simulink model "c00003M_harness"  (R2018a)
settings: Solver=FixedStepAuto  StartTime=0.0  StopTime=300  FixedStep=0.1  RelTol=1e-3
undefined symbols (not defined in the file): A1, hmax, PriorityTank, R1, R2, sigbuilder_block
(part 1 of 44)
settings Model: Creator=aarrieta  LastModifiedBy=umarkiegi

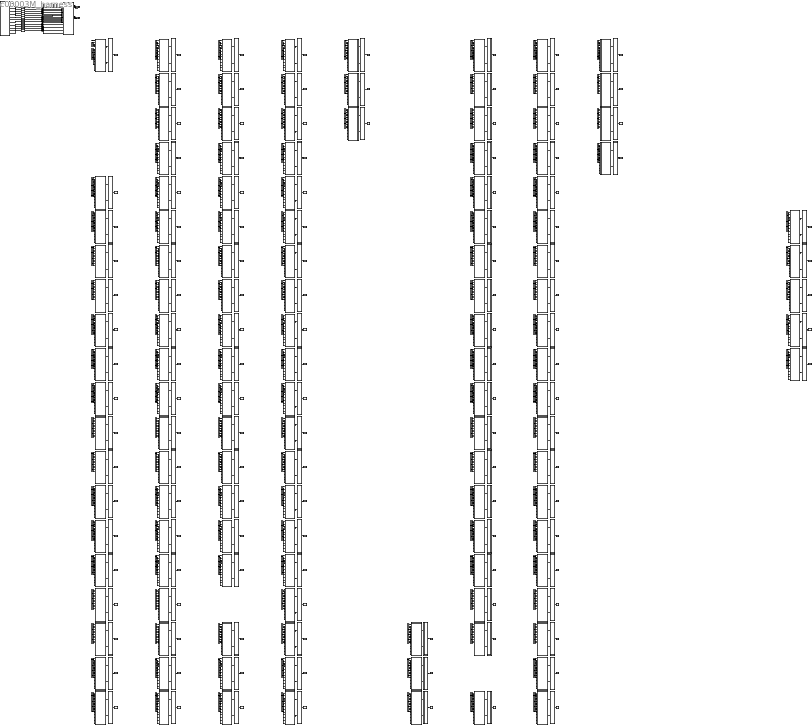
== system c00003M_harness ==
  CPSUT : Subsystem
  Eval : Subsystem
  Eval10 : Subsystem
  Eval11 : Subsystem
  Eval117 : Subsystem
  Eval118 : Subsystem
  Eval119 : Subsystem
  Eval12 : Subsystem
  Eval120 : Subsystem
  Eval121 : Subsystem
  Eval122 : Subsystem
  Eval123 : Subsystem
  Eval124 : Subsystem
  Eval125 : Subsystem
  Eval126 : Subsystem
  Eval127 : Subsystem
  Eval128 : Subsystem
  Eval129 : Subsystem
  Eval13 : Subsystem
  Eval130 : Subsystem
  Eval131 : Subsystem
  Eval132 : Subsystem
  Eval133 : Subsystem
  Eval134 : Subsystem
  Eval135 : Subsystem
  Eval136 : Subsystem
  Eval137 : Subsystem
  Eval139 : Subsystem
  Eval14 : Subsystem
  Eval140 : Subsystem
  Eval141 : Subsystem
  Eval142 : Subsystem
  Eval143 : Subsystem
  Eval144 : Subsystem
  Eval145 : Subsystem
  Eval146 : Subsystem
  Eval147 : Subsystem
  Eval148 : Subsystem
  Eval149 : Subsystem
  Eval15 : Subsystem
  Eval150 : Subsystem
  Eval151 : Subsystem
  Eval152 : Subsystem
  Eval153 : Subsystem
  Eval154 : Subsystem
  Eval155 : Subsystem
  Eval156 : Subsystem
  Eval157 : Subsystem
  Eval158 : Subsystem
  Eval159 : Subsystem
  Eval16 : Subsystem
  Eval160 : Subsystem
  Eval161 : Subsystem
  Eval162 : Subsystem
  Eval163 : Subsystem
  Eval17 : Subsystem
  Eval18 : Subsystem
  Eval19 : Subsystem
  Eval20 : Subsystem
  Eval21 : Subsystem
  Eval22 : Subsystem
  Eval225 : Subsystem
  Eval226 : Subsystem
  Eval227 : Subsystem
  Eval228 : Subsystem
  Eval229 : Subsystem
  Eval23 : Subsystem
  Eval24 : Subsystem
  Eval25 : Subsystem
  Eval26 : Subsystem
  Eval27 : Subsystem
  Eval28 : Subsystem
  Eval29 : Subsystem
  Eval30 : Subsystem
  Eval31 : Subsystem
  Eval32 : Subsystem
  Eval33 : Subsystem
  Eval34 : Subsystem
  Eval35 : Subsystem
  Eval36 : Subsystem
  Eval37 : Subsystem
  Eval38 : Subsystem
  Eval39 : Subsystem
  Eval4 : Subsystem
  Eval40 : Subsystem
  Eval41 : Subsystem
  Eval42 : Subsystem
  Eval43 : Subsystem
  Eval44 : Subsystem
  Eval45 : Subsystem
  Eval46 : Subsystem
  Eval47 : Subsystem
  Eval48 : Subsystem
  Eval49 : Subsystem
  Eval5 : Subsystem
  Eval50 : Subsystem
  Eval51 : Subsystem
  Eval52 : Subsystem
  Eval53 : Subsystem
  Eval54 : Subsystem
  Eval55 : Subsystem
  Eval57 : Subsystem
  Eval58 : Subsystem
  Eval59 : Subsystem
  Eval6 : Subsystem
  Eval60 : Subsystem
  Eval61 : Subsystem
  Eval62 : Subsystem
  Eval63 : Subsystem
  Eval64 : Subsystem
  Eval65 : Subsystem
  Eval66 : Subsystem
  Eval67 : Subsystem
  Eval68 : Subsystem
  Eval69 : Subsystem
  Eval7 : Subsystem
  Eval70 : Subsystem
  Eval71 : Subsystem
  Eval72 : Subsystem
  Eval73 : Subsystem
  Eval74 : Subsystem
  Eval75 : Subsystem
  Eval76 : Subsystem
  Eval77 : Subsystem
  Eval78 : Subsystem
  Eval79 : Subsystem
  Eval8 : Subsystem
  Eval80 : Subsystem
  Eval81 : Subsystem
  Eval82 : Subsystem
  Eval9 : Subsystem
  Inputs : Subsystem  Tag=STV Subsys  LoadFcn=sigbuilder_block('load');  StartFcn=sigbuilder_block('start');  StopFcn=sigbuilder_block('stop');  ClipboardFcn=sigbuilder_block('clipboard');  mask(Sigbuilder block){tuvar=[0:10]}
      mask init:
      | if ~strcmp(get_param(bdroot(gcb),'SimulationStatus'),'stopped'),tuvar = sigbuilder_block('maskInit'); end
      settings: CopyFcn=sigbuilder_block('copy');  DeleteFcn=sigbuilder_block('delete');  ModelCloseFcn=sigbuilder_block('modelClose');  PreSaveFcn=sigbuilder_block('preSave');  PauseFcn=sigbuilder_block('pause');  ContinueFcn=sigbuilder_block('continue');  NameChangeFcn=sigbuilder_block('namechange');  OpenFcn=sigbuilder_block('open',[276.75 163.5 675.75 486.75 ]);  CloseFcn=sigbuilder_block('close');
      mask Display: plot(0, 0, 100, 100,[2, 2, 32, 32, 2], [68, 8, 8, 68, 68],[32, 2], [38, 38], [32, 19, 2],[53, 60, 44], [32, 17, 17, 2],[16, 16, 31, 31]);txt = getActiveGroup(gcbh);text(2, 100, txt,'verticalAlignment', 'top');
  M001 : Subsystem
  M005 : Subsystem
  M006 : Subsystem
  M007 : Subsystem
  M008 : Subsystem
  M009 : Subsystem
  M010 : Subsystem
  M011 : Subsystem
  M012 : Subsystem
  M013 : Subsystem
  M014 : Subsystem
  M015 : Subsystem
  M016 : Subsystem
  M017 : Subsystem
  M018 : Subsystem
  M019 : Subsystem
  M020 : Subsystem
  M021 : Subsystem
  M022 : Subsystem
  M023 : Subsystem
  M024 : Subsystem
  M025 : Subsystem
  M026 : Subsystem
  M027 : Subsystem
  M028 : Subsystem
  M029 : Subsystem
  M030 : Subsystem
  M031 : Subsystem
  M032 : Subsystem
  M033 : Subsystem
  M034 : Subsystem
  M035 : Subsystem
  M036 : Subsystem
  M037 : Subsystem
  M038 : Subsystem
  M039 : Subsystem
  M040 : Subsystem
  M041 : Subsystem
  M042 : Subsystem
  M043 : Subsystem
  M044 : Subsystem
  M045 : Subsystem
  M046 : Subsystem
  M047 : Subsystem
  M048 : Subsystem
  M049 : Subsystem
  M050 : Subsystem
  M051 : Subsystem
  M052 : Subsystem
  M053 : Subsystem
  M054 : Subsystem
  M055 : Subsystem
  M056 : Subsystem
  M058 : Subsystem
  M059 : Subsystem
  M060 : Subsystem
  M061 : Subsystem
  M062 : Subsystem
  M063 : Subsystem
  M064 : Subsystem
  M065 : Subsystem
  M066 : Subsystem
  M067 : Subsystem
  M068 : Subsystem
  M069 : Subsystem
  M070 : Subsystem
  M071 : Subsystem
  M072 : Subsystem
  M073 : Subsystem
  M074 : Subsystem
  M075 : Subsystem
  M076 : Subsystem
  M077 : Subsystem
  M078 : Subsystem
  M079 : Subsystem
  M080 : Subsystem
  M081 : Subsystem
  M082 : Subsystem
  M083 : Subsystem
  M118 : Subsystem
  M119 : Subsystem
  M120 : Subsystem
  M121 : Subsystem
  M122 : Subsystem
  M123 : Subsystem
  M124 : Subsystem
  M125 : Subsystem
  M126 : Subsystem
  M127 : Subsystem
  M128 : Subsystem
  M129 : Subsystem
  M130 : Subsystem
  M131 : Subsystem
  M132 : Subsystem
  M133 : Subsystem
  M134 : Subsystem
  M135 : Subsystem
  M136 : Subsystem
  M137 : Subsystem
  M138 : Subsystem
  M140 : Subsystem
  M141 : Subsystem
  M142 : Subsystem
  M143 : Subsystem
  M144 : Subsystem
  M145 : Subsystem
  M146 : Subsystem
  M147 : Subsystem
  M148 : Subsystem
  M149 : Subsystem
  M150 : Subsystem
  M151 : Subsystem
  M152 : Subsystem
  M153 : Subsystem
  M154 : Subsystem
  M155 : Subsystem
  M156 : Subsystem
  M157 : Subsystem
  M158 : Subsystem
  M159 : Subsystem
  M160 : Subsystem
  M161 : Subsystem
  M162 : Subsystem
  M163 : Subsystem
  M164 : Subsystem
  M226 : Subsystem
  M227 : Subsystem
  M228 : Subsystem
  M229 : Subsystem
  M230 : Subsystem
  To Workspace : ToWorkspace  VariableName=mutant001  SampleTime=-1
  To Workspace10 : ToWorkspace  VariableName=mutant011  SampleTime=-1
  To Workspace11 : ToWorkspace  VariableName=mutant012  SampleTime=-1
  To Workspace117 : ToWorkspace  VariableName=mutant118  SampleTime=-1
  To Workspace118 : ToWorkspace  VariableName=mutant119  SampleTime=-1
  To Workspace119 : ToWorkspace  VariableName=mutant120  SampleTime=-1
  To Workspace12 : ToWorkspace  VariableName=mutant013  SampleTime=-1
  To Workspace120 : ToWorkspace  VariableName=mutant121  SampleTime=-1
  To Workspace121 : ToWorkspace  VariableName=mutant122  SampleTime=-1
  To Workspace122 : ToWorkspace  VariableName=mutant123  SampleTime=-1
  To Workspace123 : ToWorkspace  VariableName=mutant124  SampleTime=-1
  To Workspace124 : ToWorkspace  VariableName=mutant125  SampleTime=-1
  To Workspace125 : ToWorkspace  VariableName=mutant126  SampleTime=-1
  To Workspace126 : ToWorkspace  VariableName=mutant127  SampleTime=-1
  To Workspace127 : ToWorkspace  VariableName=mutant128  SampleTime=-1
  To Workspace128 : ToWorkspace  VariableName=mutant129  SampleTime=-1
  To Workspace129 : ToWorkspace  VariableName=mutant130  SampleTime=-1
  To Workspace13 : ToWorkspace  VariableName=mutant014  SampleTime=-1
  To Workspace130 : ToWorkspace  VariableName=mutant131  SampleTime=-1
  To Workspace131 : ToWorkspace  VariableName=mutant132  SampleTime=-1
  To Workspace132 : ToWorkspace  VariableName=mutant133  SampleTime=-1
  To Workspace133 : ToWorkspace  VariableName=mutant134  SampleTime=-1
  To Workspace134 : ToWorkspace  VariableName=mutant135  SampleTime=-1
  To Workspace135 : ToWorkspace  VariableName=mutant136  SampleTime=-1
  To Workspace136 : ToWorkspace  VariableName=mutant137  SampleTime=-1
  To Workspace137 : ToWorkspace  VariableName=mutant138  SampleTime=-1
  To Workspace139 : ToWorkspace  VariableName=mutant140  SampleTime=-1
  To Workspace14 : ToWorkspace  VariableName=mutant015  SampleTime=-1
  To Workspace140 : ToWorkspace  VariableName=mutant141  SampleTime=-1
  To Workspace141 : ToWorkspace  VariableName=mutant142  SampleTime=-1
  To Workspace142 : ToWorkspace  VariableName=mutant143  SampleTime=-1
  To Workspace143 : ToWorkspace  VariableName=mutant144  SampleTime=-1
  To Workspace144 : ToWorkspace  VariableName=mutant145  SampleTime=-1
  To Workspace145 : ToWorkspace  VariableName=mutant146  SampleTime=-1
  To Workspace146 : ToWorkspace  VariableName=mutant147  SampleTime=-1
  To Workspace147 : ToWorkspace  VariableName=mutant148  SampleTime=-1
  To Workspace148 : ToWorkspace  VariableName=mutant149  SampleTime=-1
  To Workspace149 : ToWorkspace  VariableName=mutant150  SampleTime=-1
  To Workspace15 : ToWorkspace  VariableName=mutant016  SampleTime=-1
  To Workspace150 : ToWorkspace  VariableName=mutant151  SampleTime=-1
  To Workspace151 : ToWorkspace  VariableName=mutant152  SampleTime=-1
  To Workspace152 : ToWorkspace  VariableName=mutant153  SampleTime=-1
  To Workspace153 : ToWorkspace  VariableName=mutant154  SampleTime=-1
  To Workspace154 : ToWorkspace  VariableName=mutant155  SampleTime=-1
  To Workspace155 : ToWorkspace  VariableName=mutant156  SampleTime=-1
  To Workspace156 : ToWorkspace  VariableName=mutant157  SampleTime=-1
  To Workspace157 : ToWorkspace  VariableName=mutant158  SampleTime=-1
  To Workspace158 : ToWorkspace  VariableName=mutant159  SampleTime=-1
  To Workspace159 : ToWorkspace  VariableName=mutant160  SampleTime=-1
  To Workspace16 : ToWorkspace  VariableName=mutant017  SampleTime=-1
  To Workspace160 : ToWorkspace  VariableName=mutant161  SampleTime=-1
  To Workspace161 : ToWorkspace  VariableName=mutant162  SampleTime=-1
  To Workspace162 : ToWorkspace  VariableName=mutant163  SampleTime=-1
  To Workspace163 : ToWorkspace  VariableName=mutant164  SampleTime=-1
  To Workspace17 : ToWorkspace  VariableName=mutant018  SampleTime=-1
  To Workspace18 : ToWorkspace  VariableName=mutant019  SampleTime=-1
  To Workspace19 : ToWorkspace  VariableName=mutant020  SampleTime=-1
  To Workspace20 : ToWorkspace  VariableName=mutant021  SampleTime=-1
  To Workspace21 : ToWorkspace  VariableName=mutant022  SampleTime=-1
  To Workspace22 : ToWorkspace  VariableName=mutant023  SampleTime=-1
  To Workspace225 : ToWorkspace  VariableName=mutant226  SampleTime=-1
  To Workspace226 : ToWorkspace  VariableName=mutant227  SampleTime=-1
  To Workspace227 : ToWorkspace  VariableName=mutant228  SampleTime=-1
  To Workspace228 : ToWorkspace  VariableName=mutant229  SampleTime=-1
  To Workspace229 : ToWorkspace  VariableName=mutant230  SampleTime=-1
  To Workspace23 : ToWorkspace  VariableName=mutant024  SampleTime=-1
  To Workspace24 : ToWorkspace  VariableName=mutant025  SampleTime=-1
  To Workspace25 : ToWorkspace  VariableName=mutant026  SampleTime=-1
  To Workspace26 : ToWorkspace  VariableName=mutant027  SampleTime=-1
  To Workspace27 : ToWorkspace  VariableName=mutant028  SampleTime=-1
  To Workspace28 : ToWorkspace  VariableName=mutant029  SampleTime=-1
  To Workspace29 : ToWorkspace  VariableName=mutant030  SampleTime=-1
  To Workspace30 : ToWorkspace  VariableName=mutant031  SampleTime=-1
  To Workspace31 : ToWorkspace  VariableName=mutant032  SampleTime=-1
  To Workspace32 : ToWorkspace  VariableName=mutant033  SampleTime=-1
  To Workspace33 : ToWorkspace  VariableName=mutant034  SampleTime=-1
  To Workspace34 : ToWorkspace  VariableName=mutant035  SampleTime=-1
  To Workspace35 : ToWorkspace  VariableName=mutant036  SampleTime=-1
  To Workspace36 : ToWorkspace  VariableName=mutant037  SampleTime=-1
  To Workspace37 : ToWorkspace  VariableName=mutant038  SampleTime=-1
  To Workspace38 : ToWorkspace  VariableName=mutant039  SampleTime=-1
  To Workspace39 : ToWorkspace  VariableName=mutant040  SampleTime=-1
  To Workspace4 : ToWorkspace  VariableName=mutant005  SampleTime=-1
  To Workspace40 : ToWorkspace  VariableName=mutant041  SampleTime=-1
  To Workspace41 : ToWorkspace  VariableName=mutant042  SampleTime=-1
  To Workspace42 : ToWorkspace  VariableName=mutant043  SampleTime=-1
  To Workspace43 : ToWorkspace  VariableName=mutant044  SampleTime=-1
  To Workspace44 : ToWorkspace  VariableName=mutant045  SampleTime=-1
  To Workspace45 : ToWorkspace  VariableName=mutant046  SampleTime=-1
  To Workspace46 : ToWorkspace  VariableName=mutant047  SampleTime=-1
  To Workspace47 : ToWorkspace  VariableName=mutant048  SampleTime=-1
  To Workspace48 : ToWorkspace  VariableName=mutant049  SampleTime=-1
  To Workspace49 : ToWorkspace  VariableName=mutant050  SampleTime=-1
  To Workspace5 : ToWorkspace  VariableName=mutant006  SampleTime=-1
  To Workspace50 : ToWorkspace  VariableName=mutant051  SampleTime=-1
  To Workspace51 : ToWorkspace  VariableName=mutant052  SampleTime=-1
  To Workspace52 : ToWorkspace  VariableName=mutant053  SampleTime=-1
  To Workspace53 : ToWorkspace  VariableName=mutant054  SampleTime=-1
  To Workspace54 : ToWorkspace  VariableName=mutant055  SampleTime=-1
  To Workspace55 : ToWorkspace  VariableName=mutant056  SampleTime=-1
  To Workspace57 : ToWorkspace  VariableName=mutant058  SampleTime=-1
  To Workspace58 : ToWorkspace  VariableName=mutant059  SampleTime=-1
  To Workspace59 : ToWorkspace  VariableName=mutant060  SampleTime=-1
  To Workspace6 : ToWorkspace  VariableName=mutant007  SampleTime=-1
  To Workspace60 : ToWorkspace  VariableName=mutant061  SampleTime=-1
  To Workspace61 : ToWorkspace  VariableName=mutant062  SampleTime=-1
  To Workspace62 : ToWorkspace  VariableName=mutant063  SampleTime=-1
  To Workspace63 : ToWorkspace  VariableName=mutant064  SampleTime=-1
  To Workspace64 : ToWorkspace  VariableName=mutant065  SampleTime=-1
  To Workspace65 : ToWorkspace  VariableName=mutant066  SampleTime=-1
  To Workspace66 : ToWorkspace  VariableName=mutant067  SampleTime=-1
  To Workspace67 : ToWorkspace  VariableName=mutant068  SampleTime=-1
  To Workspace68 : ToWorkspace  VariableName=mutant069  SampleTime=-1
  To Workspace69 : ToWorkspace  VariableName=mutant070  SampleTime=-1
  To Workspace7 : ToWorkspace  VariableName=mutant008  SampleTime=-1
  To Workspace70 : ToWorkspace  VariableName=mutant071  SampleTime=-1
  To Workspace71 : ToWorkspace  VariableName=mutant072  SampleTime=-1
  To Workspace72 : ToWorkspace  VariableName=mutant073  SampleTime=-1
  To Workspace73 : ToWorkspace  VariableName=mutant074  SampleTime=-1
  To Workspace74 : ToWorkspace  VariableName=mutant075  SampleTime=-1
  To Workspace75 : ToWorkspace  VariableName=mutant076  SampleTime=-1
  To Workspace76 : ToWorkspace  VariableName=mutant077  SampleTime=-1
  To Workspace77 : ToWorkspace  VariableName=mutant078  SampleTime=-1
  To Workspace78 : ToWorkspace  VariableName=mutant079  SampleTime=-1
  To Workspace79 : ToWorkspace  VariableName=mutant080  SampleTime=-1
  To Workspace8 : ToWorkspace  VariableName=mutant009  SampleTime=-1
  To Workspace80 : ToWorkspace  VariableName=mutant081  SampleTime=-1
  To Workspace81 : ToWorkspace  VariableName=mutant082  SampleTime=-1
  To Workspace82 : ToWorkspace  VariableName=mutant083  SampleTime=-1
  To Workspace9 : ToWorkspace  VariableName=mutant010  SampleTime=-1
  dtc_CT1 : DataTypeConversion
  dtc_CT2 : DataTypeConversion
  dtc_E1 : DataTypeConversion
  dtc_E2 : DataTypeConversion
  dtc_EB1 : DataTypeConversion
  dtc_EB2 : DataTypeConversion
  dtc_F1 : DataTypeConversion
  dtc_F2 : DataTypeConversion
  dtc_MR1 : DataTypeConversion
  dtc_MR2 : DataTypeConversion
  dtc_T1 : DataTypeConversion
  dtc_T2 : DataTypeConversion
  LL1 : Outport
  LL2 : Outport  Port=2
  tag scope: out1=global, out2=global
  wires:
  CPSUT/1(LL1) -> [out1], LL1/1
  CPSUT/2(LL2) -> [out2], LL2/1
  [in1] -> M001/1(CT1)
  [in2] -> M001/2(F1)
  [in3] -> M001/3(E1)
  [in4] -> M001/4(MR1)
  [in6] -> M001/5(EB1)
  [in7] -> M001/6(CT2)
  [in8] -> M001/7(F2)
  [in9] -> M001/8(E2)
  [in10] -> M001/9(MR2)
  [in11] -> M001/10(T2)
  [in12] -> M001/11(EB2)
  Eval/1(Out1) -> To Workspace/1
  M001/1(LL1) -> Eval/1(In1)
  M001/2(LL2) -> Eval/2(In2)
  [in1] -> M005/1(CT1)
  [in2] -> M005/2(F1)
  [in3] -> M005/3(E1)
  [in4] -> M005/4(MR1)
  [in5] -> M005/5(T1)
  [in6] -> M005/6(EB1)
  [in7] -> M005/7(CT2)
  [in8] -> M005/8(F2)
  [in9] -> M005/9(E2)
  [in10] -> M005/10(MR2)
  [in11] -> M005/11(T2)
  [in12] -> M005/12(EB2)
  M005/1(LL1) -> Eval4/1(In1)
  M005/2(LL2) -> Eval4/2(In2)
  Eval4/1(Out1) -> To Workspace4/1
  [in1] -> M006/1(CT1)
  [in2] -> M006/2(F1)
  [in3] -> M006/3(E1)
  [in4] -> M006/4(MR1)
  [in5] -> M006/5(T1)
  [in6] -> M006/6(EB1)
  [in7] -> M006/7(CT2)
  [in8] -> M006/8(F2)
  [in9] -> M006/9(E2)
  [in10] -> M006/10(MR2)
  [in11] -> M006/11(T2)
  [in12] -> M006/12(EB2)
  M006/1(LL1) -> Eval5/1(In1)
  M006/2(LL2) -> Eval5/2(In2)
  Eval5/1(Out1) -> To Workspace5/1
  [in1] -> M007/1(CT1)
  [in2] -> M007/2(F1)
  [in3] -> M007/3(E1)
  [in4] -> M007/4(MR1)
  [in5] -> M007/5(T1)
  [in6] -> M007/6(EB1)
  [in7] -> M007/7(CT2)
  [in8] -> M007/8(F2)
  [in9] -> M007/9(E2)
  [in10] -> M007/10(MR2)
  [in11] -> M007/11(T2)
  [in12] -> M007/12(EB2)
  M007/1(LL1) -> Eval6/1(In1)
  M007/2(LL2) -> Eval6/2(In2)
  Eval6/1(Out1) -> To Workspace6/1
  [in1] -> M008/1(CT1)
  [in2] -> M008/2(F1)
  [in3] -> M008/3(E1)
  [in4] -> M008/4(MR1)
  [in5] -> M008/5(T1)
  [in6] -> M008/6(EB1)
  [in7] -> M008/7(CT2)
  [in8] -> M008/8(F2)
  [in9] -> M008/9(E2)
  [in10] -> M008/10(MR2)
  [in11] -> M008/11(T2)
  [in12] -> M008/12(EB2)
  M008/1(LL1) -> Eval7/1(In1)
  M008/2(LL2) -> Eval7/2(In2)
  Eval7/1(Out1) -> To Workspace7/1
  [in1] -> M009/1(CT1)
  [in2] -> M009/2(F1)
  [in3] -> M009/3(E1)
  [in4] -> M009/4(MR1)
  [in5] -> M009/5(T1)
  [in6] -> M009/6(EB1)
  [in7] -> M009/7(CT2)
  [in8] -> M009/8(F2)
  [in9] -> M009/9(E2)
  [in10] -> M009/10(MR2)
  [in11] -> M009/11(T2)
  [in12] -> M009/12(EB2)
  M009/1(LL1) -> Eval8/1(In1)
  M009/2(LL2) -> Eval8/2(In2)
  Eval8/1(Out1) -> To Workspace8/1
  [in1] -> M010/1(CT1)
  [in2] -> M010/2(F1)
  [in3] -> M010/3(E1)
  [in4] -> M010/4(MR1)
  [in5] -> M010/5(T1)
  [in6] -> M010/6(EB1)
  [in7] -> M010/7(CT2)
  [in8] -> M010/8(F2)
  [in9] -> M010/9(E2)
  [in10] -> M010/10(MR2)
  [in11] -> M010/11(T2)
  [in12] -> M010/12(EB2)
  M010/1(LL1) -> Eval9/1(In1)
  M010/2(LL2) -> Eval9/2(In2)
  Eval9/1(Out1) -> To Workspace9/1
  [in1] -> M011/1(CT1)
  [in2] -> M011/2(F1)
  [in3] -> M011/3(E1)
  [in4] -> M011/4(MR1)
  [in5] -> M011/5(T1)
  [in6] -> M011/6(EB1)
  [in7] -> M011/7(CT2)
  [in8] -> M011/8(F2)
  [in9] -> M011/9(E2)
  [in10] -> M011/10(MR2)
  [in11] -> M011/11(T2)
  [in12] -> M011/12(EB2)
  M011/1(LL1) -> Eval10/1(In1)
  M011/2(LL2) -> Eval10/2(In2)
  Eval10/1(Out1) -> To Workspace10/1
  [in1] -> M012/1(CT1)
  [in2] -> M012/2(F1)
  [in3] -> M012/3(E1)
  [in4] -> M012/4(MR1)
  [in5] -> M012/5(T1)
  [in6] -> M012/6(EB1)
  [in7] -> M012/7(CT2)
  [in8] -> M012/8(F2)
  [in9] -> M012/9(E2)
  [in10] -> M012/10(MR2)
  [in11] -> M012/11(T2)
  [in12] -> M012/12(EB2)
  M012/1(LL1) -> Eval11/1(In1)
  M012/2(LL2) -> Eval11/2(In2)
  Eval11/1(Out1) -> To Workspace11/1
  [in1] -> M013/1(CT1)
  [in2] -> M013/2(F1)
  [in3] -> M013/3(E1)
  [in4] -> M013/4(MR1)
  [in5] -> M013/5(T1)
  [in6] -> M013/6(EB1)
  [in7] -> M013/7(CT2)
  [in8] -> M013/8(F2)
  [in9] -> M013/9(E2)
  [in10] -> M013/10(MR2)
  [in11] -> M013/11(T2)
  [in12] -> M013/12(EB2)
  M013/1(LL1) -> Eval12/1(In1)
  M013/2(LL2) -> Eval12/2(In2)
  Eval12/1(Out1) -> To Workspace12/1
  [in1] -> M014/1(CT1)
  [in2] -> M014/2(F1)
  [in3] -> M014/3(E1)
  [in4] -> M014/4(MR1)
  [in5] -> M014/5(T1)
  [in6] -> M014/6(EB1)
  [in7] -> M014/7(CT2)
  [in8] -> M014/8(F2)
  [in9] -> M014/9(E2)
  [in10] -> M014/10(MR2)
  [in11] -> M014/11(T2)
  [in12] -> M014/12(EB2)
  M014/1(LL1) -> Eval13/1(In1)
  M014/2(LL2) -> Eval13/2(In2)
  Eval13/1(Out1) -> To Workspace13/1
  [in1] -> M015/1(CT1)
  [in2] -> M015/2(F1)
  [in3] -> M015/3(E1)
  [in4] -> M015/4(MR1)
  [in5] -> M015/5(T1)
  [in6] -> M015/6(EB1)
  [in7] -> M015/7(CT2)
  [in8] -> M015/8(F2)
  [in9] -> M015/9(E2)
  [in10] -> M015/10(MR2)
  [in11] -> M015/11(T2)
  [in12] -> M015/12(EB2)
  M015/1(LL1) -> Eval14/1(In1)
  M015/2(LL2) -> Eval14/2(In2)
  Eval14/1(Out1) -> To Workspace14/1
  [in1] -> M016/1(CT1)
  [in2] -> M016/2(F1)
  [in3] -> M016/3(E1)
  [in4] -> M016/4(MR1)
  [in5] -> M016/5(T1)
  [in6] -> M016/6(EB1)
  [in7] -> M016/7(CT2)
  [in8] -> M016/8(F2)
  [in9] -> M016/9(E2)
  [in10] -> M016/10(MR2)
  [in11] -> M016/11(T2)
  [in12] -> M016/12(EB2)
  M016/1(LL1) -> Eval15/1(In1)
  M016/2(LL2) -> Eval15/2(In2)
  Eval15/1(Out1) -> To Workspace15/1
  [in1] -> M017/1(CT1)
  [in2] -> M017/2(F1)
  [in3] -> M017/3(E1)
  [in4] -> M017/4(MR1)
  [in5] -> M017/5(T1)
  [in6] -> M017/6(EB1)
  [in7] -> M017/7(CT2)
  [in8] -> M017/8(F2)
  [in9] -> M017/9(E2)
  [in10] -> M017/10(MR2)
  [in11] -> M017/11(T2)
  [in12] -> M017/12(EB2)
  M017/1(LL1) -> Eval16/1(In1)
  M017/2(LL2) -> Eval16/2(In2)
  Eval16/1(Out1) -> To Workspace16/1
  [in1] -> M018/1(CT1)
  [in2] -> M018/2(F1)
  [in3] -> M018/3(E1)
  [in4] -> M018/4(MR1)
  [in5] -> M018/5(T1)
  [in6] -> M018/6(EB1)
  [in7] -> M018/7(CT2)
  [in8] -> M018/8(F2)
  [in9] -> M018/9(E2)
  [in10] -> M018/10(MR2)
  [in11] -> M018/11(T2)
  [in12] -> M018/12(EB2)
  M018/1(LL1) -> Eval17/1(In1)
  M018/2(LL2) -> Eval17/2(In2)
  Eval17/1(Out1) -> To Workspace17/1
  [in1] -> M019/1(CT1)
  [in2] -> M019/2(F1)
  [in3] -> M019/3(E1)
  [in4] -> M019/4(MR1)
  [in5] -> M019/5(T1)
  [in6] -> M019/6(EB1)
  [in7] -> M019/7(CT2)
  [in8] -> M019/8(F2)
  [in9] -> M019/9(E2)
  [in10] -> M019/10(MR2)
  [in11] -> M019/11(T2)
  [in12] -> M019/12(EB2)
  M019/1(LL1) -> Eval18/1(In1)
  M019/2(LL2) -> Eval18/2(In2)
  Eval18/1(Out1) -> To Workspace18/1
  [in1] -> M020/1(CT1)
  [in2] -> M020/2(F1)
  [in3] -> M020/3(E1)
  [in4] -> M020/4(MR1)
  [in5] -> M020/5(T1)
  [in6] -> M020/6(EB1)
  [in7] -> M020/7(CT2)
  [in8] -> M020/8(F2)
  [in9] -> M020/9(E2)
  [in10] -> M020/10(MR2)
  [in11] -> M020/11(T2)
  [in12] -> M020/12(EB2)
  M020/1(LL1) -> Eval19/1(In1)
  M020/2(LL2) -> Eval19/2(In2)
  Eval19/1(Out1) -> To Workspace19/1
  [in1] -> M021/1(CT1)
  [in2] -> M021/2(F1)
  [in3] -> M021/3(E1)
  [in4] -> M021/4(MR1)
  [in5] -> M021/5(T1)
  [in6] -> M021/6(EB1)
  [in7] -> M021/7(CT2)
  [in8] -> M021/8(F2)
  [in9] -> M021/9(E2)
  [in10] -> M021/10(MR2)
  [in11] -> M021/11(T2)
  [in12] -> M021/12(EB2)
  M021/1(LL1) -> Eval20/1(In1)
  M021/2(LL2) -> Eval20/2(In2)
  Eval20/1(Out1) -> To Workspace20/1
  [in1] -> M022/1(CT1)
  [in2] -> M022/2(F1)
  [in3] -> M022/3(E1)
  [in4] -> M022/4(MR1)
  [in5] -> M022/5(T1)
  [in6] -> M022/6(EB1)
  [in7] -> M022/7(CT2)
  [in8] -> M022/8(F2)
  [in9] -> M022/9(E2)
  [in10] -> M022/10(MR2)
  [in11] -> M022/11(T2)
  [in12] -> M022/12(EB2)
  M022/1(LL1) -> Eval21/1(In1)
  M022/2(LL2) -> Eval21/2(In2)
  Eval21/1(Out1) -> To Workspace21/1
  [in1] -> M023/1(CT1)
  [in2] -> M023/2(F1)
  [in3] -> M023/3(E1)
  [in4] -> M023/4(MR1)
  [in5] -> M023/5(T1)
  [in6] -> M023/6(EB1)
  [in7] -> M023/7(CT2)
  [in8] -> M023/8(F2)
  [in9] -> M023/9(E2)
  [in10] -> M023/10(MR2)
  [in11] -> M023/11(T2)
  [in12] -> M023/12(EB2)
  M023/1(LL1) -> Eval22/1(In1)
  M023/2(LL2) -> Eval22/2(In2)
  Eval22/1(Out1) -> To Workspace22/1
  [in1] -> M024/1(CT1)
  [in2] -> M024/2(F1)
  [in3] -> M024/3(E1)
  [in4] -> M024/4(MR1)
  [in5] -> M024/5(T1)
  [in6] -> M024/6(EB1)
  [in7] -> M024/7(CT2)
  [in8] -> M024/8(F2)
  [in9] -> M024/9(E2)
  [in10] -> M024/10(MR2)
  [in11] -> M024/11(T2)
  [in12] -> M024/12(EB2)
  M024/1(LL1) -> Eval23/1(In1)
  M024/2(LL2) -> Eval23/2(In2)
  Eval23/1(Out1) -> To Workspace23/1
  [in1] -> M025/1(CT1)
  [in2] -> M025/2(F1)
  [in3] -> M025/3(E1)
  [in4] -> M025/4(MR1)
  [in5] -> M025/5(T1)
  [in6] -> M025/6(EB1)
  [in7] -> M025/7(CT2)
  [in8] -> M025/8(F2)
  [in9] -> M025/9(E2)
  [in10] -> M025/10(MR2)
  [in11] -> M025/11(T2)
  [in12] -> M025/12(EB2)
  M025/1(LL1) -> Eval24/1(In1)
  M025/2(LL2) -> Eval24/2(In2)
  Eval24/1(Out1) -> To Workspace24/1
  [in1] -> M026/1(CT1)
  [in2] -> M026/2(F1)
  [in3] -> M026/3(E1)
  [in4] -> M026/4(MR1)
  [in5] -> M026/5(T1)
  [in6] -> M026/6(EB1)
  [in7] -> M026/7(CT2)
  [in8] -> M026/8(F2)
  [in9] -> M026/9(E2)
  [in10] -> M026/10(MR2)
  [in11] -> M026/11(T2)
  [in12] -> M026/12(EB2)
  M026/1(LL1) -> Eval25/1(In1)
  M026/2(LL2) -> Eval25/2(In2)
  Eval25/1(Out1) -> To Workspace25/1
  [in1] -> M027/1(CT1)
  [in2] -> M027/2(F1)
  [in3] -> M027/3(E1)
  [in4] -> M027/4(MR1)
  [in5] -> M027/5(T1)
  [in6] -> M027/6(EB1)
  [in7] -> M027/7(CT2)
  [in8] -> M027/8(F2)
  [in9] -> M027/9(E2)
  [in10] -> M027/10(MR2)
  [in11] -> M027/11(T2)
  [in12] -> M027/12(EB2)
  M027/1(LL1) -> Eval26/1(In1)
  M027/2(LL2) -> Eval26/2(In2)
  Eval26/1(Out1) -> To Workspace26/1
  [in1] -> M028/1(CT1)
  [in2] -> M028/2(F1)
  [in3] -> M028/3(E1)
  [in4] -> M028/4(MR1)
  [in5] -> M028/5(T1)
  [in6] -> M028/6(EB1)
  [in7] -> M028/7(CT2)
  [in8] -> M028/8(F2)
  [in9] -> M028/9(E2)
  [in10] -> M028/10(MR2)
  [in11] -> M028/11(T2)
  [in12] -> M028/12(EB2)
  M028/1(LL1) -> Eval27/1(In1)
  M028/2(LL2) -> Eval27/2(In2)
  Eval27/1(Out1) -> To Workspace27/1
  [in1] -> M029/1(CT1)
  [in2] -> M029/2(F1)
  [in3] -> M029/3(E1)
  [in4] -> M029/4(MR1)
  [in5] -> M029/5(T1)
  [in6] -> M029/6(EB1)
  [in7] -> M029/7(CT2)
  [in8] -> M029/8(F2)
  [in9] -> M029/9(E2)
  [in10] -> M029/10(MR2)
  [in11] -> M029/11(T2)
  [in12] -> M029/12(EB2)
  M029/1(LL1) -> Eval28/1(In1)
  M029/2(LL2) -> Eval28/2(In2)
  Eval28/1(Out1) -> To Workspace28/1
  [in1] -> M030/1(CT1)
  [in2] -> M030/2(F1)
  [in3] -> M030/3(E1)
  [in4] -> M030/4(MR1)
  [in5] -> M030/5(T1)
  [in6] -> M030/6(EB1)
  [in7] -> M030/7(CT2)
  [in8] -> M030/8(F2)
  [in9] -> M030/9(E2)
  [in10] -> M030/10(MR2)
  [in11] -> M030/11(T2)
  [in12] -> M030/12(EB2)
  M030/1(LL1) -> Eval29/1(In1)
  M030/2(LL2) -> Eval29/2(In2)
  Eval29/1(Out1) -> To Workspace29/1
  [in1] -> M031/1(CT1)
  [in2] -> M031/2(F1)
  [in3] -> M031/3(E1)
  [in4] -> M031/4(MR1)
  [in5] -> M031/5(T1)
  [in6] -> M031/6(EB1)
  [in7] -> M031/7(CT2)
  [in8] -> M031/8(F2)
  [in9] -> M031/9(E2)
  [in10] -> M031/10(MR2)
  [in11] -> M031/11(T2)
  [in12] -> M031/12(EB2)
  M031/1(LL1) -> Eval30/1(In1)
  M031/2(LL2) -> Eval30/2(In2)
  Eval30/1(Out1) -> To Workspace30/1
  [in1] -> M032/1(CT1)
  [in2] -> M032/2(F1)
  [in3] -> M032/3(E1)
  [in4] -> M032/4(MR1)
  [in5] -> M032/5(T1)
  [in6] -> M032/6(EB1)
  [in7] -> M032/7(CT2)
  [in8] -> M032/8(F2)
  [in9] -> M032/9(E2)
  [in10] -> M032/10(MR2)
  [in11] -> M032/11(T2)
  [in12] -> M032/12(EB2)
  M032/1(LL1) -> Eval31/1(In1)
  M032/2(LL2) -> Eval31/2(In2)
  Eval31/1(Out1) -> To Workspace31/1
  [in1] -> M033/1(CT1)
  [in2] -> M033/2(F1)
  [in3] -> M033/3(E1)
  [in4] -> M033/4(MR1)
  [in5] -> M033/5(T1)
  [in6] -> M033/6(EB1)
  [in7] -> M033/7(CT2)
  [in8] -> M033/8(F2)
  [in9] -> M033/9(E2)
  [in10] -> M033/10(MR2)
  [in11] -> M033/11(T2)
  [in12] -> M033/12(EB2)
  M033/1(LL1) -> Eval32/1(In1)
  M033/2(LL2) -> Eval32/2(In2)
  Eval32/1(Out1) -> To Workspace32/1
  [in1] -> M034/1(CT1)
  [in2] -> M034/2(F1)
  [in3] -> M034/3(E1)
  [in4] -> M034/4(MR1)
  [in5] -> M034/5(T1)
  [in6] -> M034/6(EB1)
  [in7] -> M034/7(CT2)
  [in8] -> M034/8(F2)
  [in9] -> M034/9(E2)
  [in10] -> M034/10(MR2)
  [in11] -> M034/11(T2)
  [in12] -> M034/12(EB2)
  M034/1(LL1) -> Eval33/1(In1)
  M034/2(LL2) -> Eval33/2(In2)
  Eval33/1(Out1) -> To Workspace33/1
  [in1] -> M035/1(CT1)
  [in2] -> M035/2(F1)
  [in3] -> M035/3(E1)
  [in4] -> M035/4(MR1)
  [in5] -> M035/5(T1)
  [in6] -> M035/6(EB1)
  [in7] -> M035/7(CT2)
  [in8] -> M035/8(F2)
  [in9] -> M035/9(E2)
  [in10] -> M035/10(MR2)
  [in11] -> M035/11(T2)
  [in12] -> M035/12(EB2)
  M035/1(LL1) -> Eval34/1(In1)
  M035/2(LL2) -> Eval34/2(In2)
  Eval34/1(Out1) -> To Workspace34/1
  [in1] -> M036/1(CT1)
  [in2] -> M036/2(F1)
  [in3] -> M036/3(E1)
  [in4] -> M036/4(MR1)
  [in5] -> M036/5(T1)
  [in6] -> M036/6(EB1)
  [in7] -> M036/7(CT2)
  [in8] -> M036/8(F2)
  [in9] -> M036/9(E2)
  [in10] -> M036/10(MR2)
  [in11] -> M036/11(T2)
  [in12] -> M036/12(EB2)
  M036/1(LL1) -> Eval35/1(In1)
  M036/2(LL2) -> Eval35/2(In2)
  Eval35/1(Out1) -> To Workspace35/1
  [in1] -> M037/1(CT1)
  [in2] -> M037/2(F1)
  [in3] -> M037/3(E1)
  [in4] -> M037/4(MR1)
  [in5] -> M037/5(T1)
  [in6] -> M037/6(EB1)
  [in7] -> M037/7(CT2)
  [in8] -> M037/8(F2)
  [in9] -> M037/9(E2)
  [in10] -> M037/10(MR2)
  [in11] -> M037/11(T2)
  [in12] -> M037/12(EB2)
  M037/1(LL1) -> Eval36/1(In1)
  M037/2(LL2) -> Eval36/2(In2)
  Eval36/1(Out1) -> To Workspace36/1
  [in1] -> M038/1(CT1)
  [in2] -> M038/2(F1)
  [in3] -> M038/3(E1)
  [in4] -> M038/4(MR1)
  [in5] -> M038/5(T1)
  [in6] -> M038/6(EB1)
  [in7] -> M038/7(CT2)
  [in8] -> M038/8(F2)
  [in9] -> M038/9(E2)
  [in10] -> M038/10(MR2)
  [in11] -> M038/11(T2)
  [in12] -> M038/12(EB2)
  M038/1(LL1) -> Eval37/1(In1)
  M038/2(LL2) -> Eval37/2(In2)
  Eval37/1(Out1) -> To Workspace37/1
  [in1] -> M039/1(CT1)
  [in2] -> M039/2(F1)
  [in3] -> M039/3(E1)
  [in4] -> M039/4(MR1)
  [in5] -> M039/5(T1)
  [in6] -> M039/6(EB1)
  [in7] -> M039/7(CT2)
  [in8] -> M039/8(F2)
  [in9] -> M039/9(E2)
  [in10] -> M039/10(MR2)
  [in11] -> M039/11(T2)
  [in12] -> M039/12(EB2)
  M039/1(LL1) -> Eval38/1(In1)
  M039/2(LL2) -> Eval38/2(In2)
  Eval38/1(Out1) -> To Workspace38/1
  [in1] -> M040/1(CT1)
  [in2] -> M040/2(F1)
  [in3] -> M040/3(E1)
  [in4] -> M040/4(MR1)
  [in5] -> M040/5(T1)
  [in6] -> M040/6(EB1)
  [in7] -> M040/7(CT2)
  [in8] -> M040/8(F2)
  [in9] -> M040/9(E2)
  [in10] -> M040/10(MR2)
  [in11] -> M040/11(T2)
  [in12] -> M040/12(EB2)
  M040/1(LL1) -> Eval39/1(In1)
  M040/2(LL2) -> Eval39/2(In2)
  Eval39/1(Out1) -> To Workspace39/1
  [in1] -> M041/1(CT1)
  [in2] -> M041/2(F1)
  [in3] -> M041/3(E1)
  [in4] -> M041/4(MR1)
  [in5] -> M041/5(T1)
  [in6] -> M041/6(EB1)
  [in7] -> M041/7(CT2)
  [in8] -> M041/8(F2)
  [in9] -> M041/9(E2)
  [in10] -> M041/10(MR2)
  [in11] -> M041/11(T2)
  [in12] -> M041/12(EB2)
  M041/1(LL1) -> Eval40/1(In1)
  M041/2(LL2) -> Eval40/2(In2)
  Eval40/1(Out1) -> To Workspace40/1
  [in1] -> M042/1(CT1)
  [in2] -> M042/2(F1)
  [in3] -> M042/3(E1)
  [in4] -> M042/4(MR1)
  [in5] -> M042/5(T1)
  [in6] -> M042/6(EB1)
  [in7] -> M042/7(CT2)
  [in8] -> M042/8(F2)
  [in9] -> M042/9(E2)
  [in10] -> M042/10(MR2)
  [in11] -> M042/11(T2)
  [in12] -> M042/12(EB2)
  M042/1(LL1) -> Eval41/1(In1)
  M042/2(LL2) -> Eval41/2(In2)
  Eval41/1(Out1) -> To Workspace41/1
  [in1] -> M043/1(CT1)
  [in2] -> M043/2(F1)
  [in3] -> M043/3(E1)
  [in4] -> M043/4(MR1)
  [in5] -> M043/5(T1)
  [in6] -> M043/6(EB1)
  [in7] -> M043/7(CT2)
  [in8] -> M043/8(F2)
  [in9] -> M043/9(E2)
  [in10] -> M043/10(MR2)
  [in11] -> M043/11(T2)
  [in12] -> M043/12(EB2)
  M043/1(LL1) -> Eval42/1(In1)
  M043/2(LL2) -> Eval42/2(In2)
  Eval42/1(Out1) -> To Workspace42/1
  [in1] -> M044/1(CT1)
  [in2] -> M044/2(F1)
  [in3] -> M044/3(E1)
  [in4] -> M044/4(MR1)
  [in5] -> M044/5(T1)
  [in6] -> M044/6(EB1)
  [in7] -> M044/7(CT2)
  [in8] -> M044/8(F2)
  [in9] -> M044/9(E2)
  [in10] -> M044/10(MR2)
  [in11] -> M044/11(T2)
  [in12] -> M044/12(EB2)
  M044/1(LL1) -> Eval43/1(In1)
  M044/2(LL2) -> Eval43/2(In2)
  Eval43/1(Out1) -> To Workspace43/1
  [in1] -> M045/1(CT1)
  [in2] -> M045/2(F1)
  [in3] -> M045/3(E1)
  [in4] -> M045/4(MR1)
  [in5] -> M045/5(T1)
  [in6] -> M045/6(EB1)
  [in7] -> M045/7(CT2)
  [in8] -> M045/8(F2)
  [in9] -> M045/9(E2)
  [in10] -> M045/10(MR2)
  [in11] -> M045/11(T2)
  [in12] -> M045/12(EB2)
  M045/1(LL1) -> Eval44/1(In1)
  M045/2(LL2) -> Eval44/2(In2)
  Eval44/1(Out1) -> To Workspace44/1
  [in1] -> M046/1(CT1)
  [in2] -> M046/2(F1)
  [in3] -> M046/3(E1)
  [in4] -> M046/4(MR1)
  [in5] -> M046/5(T1)
  [in6] -> M046/6(EB1)
  [in7] -> M046/7(CT2)
  [in8] -> M046/8(F2)
  [in9] -> M046/9(E2)
  [in10] -> M046/10(MR2)
  [in11] -> M046/11(T2)
  [in12] -> M046/12(EB2)
  M046/1(LL1) -> Eval45/1(In1)
  M046/2(LL2) -> Eval45/2(In2)
  Eval45/1(Out1) -> To Workspace45/1
  [in1] -> M047/1(CT1)
  [in2] -> M047/2(F1)
  [in3] -> M047/3(E1)
  [in4] -> M047/4(MR1)
  [in5] -> M047/5(T1)
  [in6] -> M047/6(EB1)
  [in7] -> M047/7(CT2)
  [in8] -> M047/8(F2)
  [in9] -> M047/9(E2)
  [in10] -> M047/10(MR2)
  [in11] -> M047/11(T2)
  [in12] -> M047/12(EB2)
  M047/1(LL1) -> Eval46/1(In1)
  M047/2(LL2) -> Eval46/2(In2)
  Eval46/1(Out1) -> To Workspace46/1
  [in1] -> M048/1(CT1)
  [in2] -> M048/2(F1)
  [in3] -> M048/3(E1)
  [in4] -> M048/4(MR1)
  [in5] -> M048/5(T1)
  [in6] -> M048/6(EB1)
  [in7] -> M048/7(CT2)
  [in8] -> M048/8(F2)
  [in9] -> M048/9(E2)
  [in10] -> M048/10(MR2)
  [in11] -> M048/11(T2)
  [in12] -> M048/12(EB2)
  M048/1(LL1) -> Eval47/1(In1)
  M048/2(LL2) -> Eval47/2(In2)
  Eval47/1(Out1) -> To Workspace47/1
  [in1] -> M049/1(CT1)
  [in2] -> M049/2(F1)
  [in3] -> M049/3(E1)
  [in4] -> M049/4(MR1)
  [in5] -> M049/5(T1)
  [in6] -> M049/6(EB1)
  [in7] -> M049/7(CT2)
  [in8] -> M049/8(F2)
  [in9] -> M049/9(E2)
  [in10] -> M049/10(MR2)
  [in11] -> M049/11(T2)
  [in12] -> M049/12(EB2)
  M049/1(LL1) -> Eval48/1(In1)
  M049/2(LL2) -> Eval48/2(In2)
  Eval48/1(Out1) -> To Workspace48/1
  [in1] -> M050/1(CT1)
  [in2] -> M050/2(F1)
  [in3] -> M050/3(E1)
  [in4] -> M050/4(MR1)
  [in5] -> M050/5(T1)
  [in6] -> M050/6(EB1)
  [in7] -> M050/7(CT2)
  [in8] -> M050/8(F2)
  [in9] -> M050/9(E2)
  [in10] -> M050/10(MR2)
  [in11] -> M050/11(T2)
  [in12] -> M050/12(EB2)
  M050/1(LL1) -> Eval49/1(In1)
  M050/2(LL2) -> Eval49/2(In2)
  Eval49/1(Out1) -> To Workspace49/1
  [in1] -> M051/1(CT1)
  [in2] -> M051/2(F1)
  [in3] -> M051/3(E1)
  [in4] -> M051/4(MR1)
  [in5] -> M051/5(T1)
  [in6] -> M051/6(EB1)
  [in7] -> M051/7(CT2)
  [in8] -> M051/8(F2)
  [in9] -> M051/9(E2)
  [in10] -> M051/10(MR2)
  [in11] -> M051/11(T2)
  [in12] -> M051/12(EB2)
  M051/1(LL1) -> Eval50/1(In1)
  M051/2(LL2) -> Eval50/2(In2)
  Eval50/1(Out1) -> To Workspace50/1
  [in1] -> M052/1(CT1)
  [in2] -> M052/2(F1)
  [in3] -> M052/3(E1)
  [in4] -> M052/4(MR1)
  [in5] -> M052/5(T1)
  [in6] -> M052/6(EB1)
  [in7] -> M052/7(CT2)
  [in8] -> M052/8(F2)
  [in9] -> M052/9(E2)
  [in10] -> M052/10(MR2)
  [in11] -> M052/11(T2)
  [in12] -> M052/12(EB2)
  M052/1(LL1) -> Eval51/1(In1)
  M052/2(LL2) -> Eval51/2(In2)
  Eval51/1(Out1) -> To Workspace51/1
  [in1] -> M053/1(CT1)
  [in2] -> M053/2(F1)
  [in3] -> M053/3(E1)
  [in4] -> M053/4(MR1)
  [in5] -> M053/5(T1)
  [in6] -> M053/6(EB1)
  [in7] -> M053/7(CT2)
  [in8] -> M053/8(F2)
  [in9] -> M053/9(E2)
  [in10] -> M053/10(MR2)
  [in11] -> M053/11(T2)
  [in12] -> M053/12(EB2)
  M053/1(LL1) -> Eval52/1(In1)
  M053/2(LL2) -> Eval52/2(In2)
  Eval52/1(Out1) -> To Workspace52/1
  [in1] -> M054/1(CT1)
  [in2] -> M054/2(F1)
  [in3] -> M054/3(E1)
  [in4] -> M054/4(MR1)
  [in5] -> M054/5(T1)
  [in6] -> M054/6(EB1)
  [in7] -> M054/7(CT2)
  [in8] -> M054/8(F2)
  [in9] -> M054/9(E2)
  [in10] -> M054/10(MR2)
  [in11] -> M054/11(T2)
  [in12] -> M054/12(EB2)
  M054/1(LL1) -> Eval53/1(In1)
  M054/2(LL2) -> Eval53/2(In2)
  Eval53/1(Out1) -> To Workspace53/1
  [in1] -> M055/1(CT1)
  [in2] -> M055/2(F1)
  [in3] -> M055/3(E1)
  [in4] -> M055/4(MR1)
  [in5] -> M055/5(T1)
  [in6] -> M055/6(EB1)
  [in7] -> M055/7(CT2)
  [in8] -> M055/8(F2)
  [in9] -> M055/9(E2)
  [in10] -> M055/10(MR2)
  [in11] -> M055/11(T2)
  [in12] -> M055/12(EB2)
  M055/1(LL1) -> Eval54/1(In1)
  M055/2(LL2) -> Eval54/2(In2)
  Eval54/1(Out1) -> To Workspace54/1
  [in1] -> M056/1(CT1)
  [in2] -> M056/2(F1)
  [in3] -> M056/3(E1)
  [in4] -> M056/4(MR1)
  [in5] -> M056/5(T1)
  [in6] -> M056/6(EB1)
  [in7] -> M056/7(CT2)
  [in8] -> M056/8(F2)
  [in9] -> M056/9(E2)
  [in10] -> M056/10(MR2)
  [in11] -> M056/11(T2)
  [in12] -> M056/12(EB2)
  M056/1(LL1) -> Eval55/1(In1)
  M056/2(LL2) -> Eval55/2(In2)
  Eval55/1(Out1) -> To Workspace55/1
  [in1] -> M058/1(CT1)
  [in2] -> M058/2(F1)
  [in3] -> M058/3(E1)
  [in4] -> M058/4(MR1)
  [in5] -> M058/5(T1)
  [in6] -> M058/6(EB1)
  [in7] -> M058/7(CT2)
  [in8] -> M058/8(F2)
  [in9] -> M058/9(E2)
  [in10] -> M058/10(MR2)
  [in11] -> M058/11(T2)
  [in12] -> M058/12(EB2)
  M058/1(LL1) -> Eval57/1(In1)
  M058/2(LL2) -> Eval57/2(In2)
  Eval57/1(Out1) -> To Workspace57/1
  [in1] -> M059/1(CT1)
  [in2] -> M059/2(F1)
  [in3] -> M059/3(E1)
  [in4] -> M059/4(MR1)
  [in5] -> M059/5(T1)
  [in6] -> M059/6(EB1)
  [in7] -> M059/7(CT2)
  [in8] -> M059/8(F2)
  [in9] -> M059/9(E2)
  [in10] -> M059/10(MR2)
  [in11] -> M059/11(T2)
  [in12] -> M059/12(EB2)
  M059/1(LL1) -> Eval58/1(In1)
  M059/2(LL2) -> Eval58/2(In2)
  Eval58/1(Out1) -> To Workspace58/1
  [in1] -> M060/1(CT1)
  [in2] -> M060/2(F1)
  [in3] -> M060/3(E1)
  [in4] -> M060/4(MR1)
  [in5] -> M060/5(T1)
  [in6] -> M060/6(EB1)
  [in7] -> M060/7(CT2)
  [in8] -> M060/8(F2)
  [in9] -> M060/9(E2)
  [in10] -> M060/10(MR2)
  [in11] -> M060/11(T2)
  [in12] -> M060/12(EB2)
  M060/1(LL1) -> Eval59/1(In1)
  M060/2(LL2) -> Eval59/2(In2)
  Eval59/1(Out1) -> To Workspace59/1
  [in1] -> M061/1(CT1)
  [in2] -> M061/2(F1)
  [in3] -> M061/3(E1)
  [in4] -> M061/4(MR1)
  [in5] -> M061/5(T1)
  [in6] -> M061/6(EB1)
  [in7] -> M061/7(CT2)
  [in8] -> M061/8(F2)
  [in9] -> M061/9(E2)
  [in10] -> M061/10(MR2)
  [in11] -> M061/11(T2)
  [in12] -> M061/12(EB2)
  M061/1(LL1) -> Eval60/1(In1)
  M061/2(LL2) -> Eval60/2(In2)
  Eval60/1(Out1) -> To Workspace60/1
  [in1] -> M062/1(CT1)
  [in2] -> M062/2(F1)
  [in3] -> M062/3(E1)
  [in4] -> M062/4(MR1)
  [in5] -> M062/5(T1)
  [in6] -> M062/6(EB1)
  [in7] -> M062/7(CT2)
  [in8] -> M062/8(F2)
  [in9] -> M062/9(E2)
  [in10] -> M062/10(MR2)
  [in11] -> M062/11(T2)
  [in12] -> M062/12(EB2)
  M062/1(LL1) -> Eval61/1(In1)
  M062/2(LL2) -> Eval61/2(In2)
  Eval61/1(Out1) -> To Workspace61/1
  [in1] -> M063/1(CT1)
  [in2] -> M063/2(F1)
  [in3] -> M063/3(E1)
  [in4] -> M063/4(MR1)
  [in5] -> M063/5(T1)
  [in6] -> M063/6(EB1)
  [in7] -> M063/7(CT2)
  [in8] -> M063/8(F2)
  [in9] -> M063/9(E2)
  [in10] -> M063/10(MR2)
  [in11] -> M063/11(T2)
  [in12] -> M063/12(EB2)
  M063/1(LL1) -> Eval62/1(In1)
  M063/2(LL2) -> Eval62/2(In2)
  Eval62/1(Out1) -> To Workspace62/1
  [in1] -> M064/1(CT1)
  [in2] -> M064/2(F1)
  [in3] -> M064/3(E1)
  [in4] -> M064/4(MR1)
  [in5] -> M064/5(T1)
  [in6] -> M064/6(EB1)
  [in7] -> M064/7(CT2)
  [in8] -> M064/8(F2)
  [in9] -> M064/9(E2)
  [in10] -> M064/10(MR2)
  [in11] -> M064/11(T2)
  [in12] -> M064/12(EB2)
  M064/1(LL1) -> Eval63/1(In1)
  M064/2(LL2) -> Eval63/2(In2)
  Eval63/1(Out1) -> To Workspace63/1
  [in1] -> M065/1(CT1)
  [in2] -> M065/2(F1)
  [in3] -> M065/3(E1)
  [in4] -> M065/4(MR1)
  [in5] -> M065/5(T1)
  [in6] -> M065/6(EB1)
  [in7] -> M065/7(CT2)
  [in8] -> M065/8(F2)
  [in9] -> M065/9(E2)
  [in10] -> M065/10(MR2)
  [in11] -> M065/11(T2)
  [in12] -> M065/12(EB2)
  M065/1(LL1) -> Eval64/1(In1)
  M065/2(LL2) -> Eval64/2(In2)
  Eval64/1(Out1) -> To Workspace64/1
  [in1] -> M066/1(CT1)
  [in2] -> M066/2(F1)
  [in3] -> M066/3(E1)
  [in4] -> M066/4(MR1)
  [in5] -> M066/5(T1)
  [in6] -> M066/6(EB1)
  [in7] -> M066/7(CT2)
  [in8] -> M066/8(F2)
  [in9] -> M066/9(E2)
  [in10] -> M066/10(MR2)
  [in11] -> M066/11(T2)
  [in12] -> M066/12(EB2)
  M066/1(LL1) -> Eval65/1(In1)
  M066/2(LL2) -> Eval65/2(In2)
  Eval65/1(Out1) -> To Workspace65/1
  [in1] -> M067/1(CT1)
  [in2] -> M067/2(F1)
  [in3] -> M067/3(E1)
  [in4] -> M067/4(MR1)
  [in5] -> M067/5(T1)
  [in6] -> M067/6(EB1)
  [in7] -> M067/7(CT2)
  [in8] -> M067/8(F2)
  [in9] -> M067/9(E2)
  [in10] -> M067/10(MR2)
  [in11] -> M067/11(T2)
  [in12] -> M067/12(EB2)
  M067/1(LL1) -> Eval66/1(In1)
  M067/2(LL2) -> Eval66/2(In2)
  Eval66/1(Out1) -> To Workspace66/1
  [in1] -> M068/1(CT1)
  [in2] -> M068/2(F1)
  [in3] -> M068/3(E1)
  [in4] -> M068/4(MR1)
  [in5] -> M068/5(T1)
  [in6] -> M068/6(EB1)
  [in7] -> M068/7(CT2)
  [in8] -> M068/8(F2)
  [in9] -> M068/9(E2)
  [in10] -> M068/10(MR2)
  [in11] -> M068/11(T2)
  [in12] -> M068/12(EB2)
  M068/1(LL1) -> Eval67/1(In1)
  M068/2(LL2) -> Eval67/2(In2)
  Eval67/1(Out1) -> To Workspace67/1
  [in1] -> M069/1(CT1)
  [in2] -> M069/2(F1)
  [in3] -> M069/3(E1)
  [in4] -> M069/4(MR1)
  [in5] -> M069/5(T1)
  [in6] -> M069/6(EB1)
  [in7] -> M069/7(CT2)
  [in8] -> M069/8(F2)
  [in9] -> M069/9(E2)
  [in10] -> M069/10(MR2)
  [in11] -> M069/11(T2)
  [in12] -> M069/12(EB2)
  M069/1(LL1) -> Eval68/1(In1)
  M069/2(LL2) -> Eval68/2(In2)
  Eval68/1(Out1) -> To Workspace68/1
  [in1] -> M070/1(CT1)
  [in2] -> M070/2(F1)
  [in3] -> M070/3(E1)
  [in4] -> M070/4(MR1)
  [in5] -> M070/5(T1)
  [in6] -> M070/6(EB1)
  [in7] -> M070/7(CT2)
  [in8] -> M070/8(F2)
  [in9] -> M070/9(E2)
  [in10] -> M070/10(MR2)
  [in11] -> M070/11(T2)
  [in12] -> M070/12(EB2)
  M070/1(LL1) -> Eval69/1(In1)
  M070/2(LL2) -> Eval69/2(In2)
  Eval69/1(Out1) -> To Workspace69/1
  [in1] -> M071/1(CT1)
  [in2] -> M071/2(F1)
  [in3] -> M071/3(E1)
  [in4] -> M071/4(MR1)
  [in5] -> M071/5(T1)
  [in6] -> M071/6(EB1)
  [in7] -> M071/7(CT2)
  [in8] -> M071/8(F2)
  [in9] -> M071/9(E2)
  [in10] -> M071/10(MR2)
  [in11] -> M071/11(T2)
  [in12] -> M071/12(EB2)
  M071/1(LL1) -> Eval70/1(In1)
  M071/2(LL2) -> Eval70/2(In2)
  Eval70/1(Out1) -> To Workspace70/1
  [in1] -> M072/1(CT1)
  [in2] -> M072/2(F1)
  [in3] -> M072/3(E1)
  [in4] -> M072/4(MR1)
  [in5] -> M072/5(T1)
  [in6] -> M072/6(EB1)
  [in7] -> M072/7(CT2)
  [in8] -> M072/8(F2)
  [in9] -> M072/9(E2)
  [in10] -> M072/10(MR2)
  [in11] -> M072/11(T2)
  [in12] -> M072/12(EB2)
  M072/1(LL1) -> Eval71/1(In1)
  M072/2(LL2) -> Eval71/2(In2)
  Eval71/1(Out1) -> To Workspace71/1
  [in1] -> M073/1(CT1)
  [in2] -> M073/2(F1)
  [in3] -> M073/3(E1)
  [in4] -> M073/4(MR1)
  [in5] -> M073/5(T1)
  [in6] -> M073/6(EB1)
  [in7] -> M073/7(CT2)
  [in8] -> M073/8(F2)
  [in9] -> M073/9(E2)
  [in10] -> M073/10(MR2)
  [in11] -> M073/11(T2)
  [in12] -> M073/12(EB2)
  M073/1(LL1) -> Eval72/1(In1)
  M073/2(LL2) -> Eval72/2(In2)
  Eval72/1(Out1) -> To Workspace72/1
  [in1] -> M074/1(CT1)
  [in2] -> M074/2(F1)
  [in3] -> M074/3(E1)
  [in4] -> M074/4(MR1)
  [in5] -> M074/5(T1)
  [in6] -> M074/6(EB1)
  [in7] -> M074/7(CT2)
  [in8] -> M074/8(F2)
  [in9] -> M074/9(E2)
  [in10] -> M074/10(MR2)
  [in11] -> M074/11(T2)
  [in12] -> M074/12(EB2)
  M074/1(LL1) -> Eval73/1(In1)
  M074/2(LL2) -> Eval73/2(In2)
  Eval73/1(Out1) -> To Workspace73/1
  [in1] -> M075/1(CT1)
  [in2] -> M075/2(F1)
  [in3] -> M075/3(E1)
  [in4] -> M075/4(MR1)
  [in5] -> M075/5(T1)
  [in6] -> M075/6(EB1)
  [in7] -> M075/7(CT2)
  [in8] -> M075/8(F2)
  [in9] -> M075/9(E2)
  [in10] -> M075/10(MR2)
  [in11] -> M075/11(T2)
  [in12] -> M075/12(EB2)
  M075/1(LL1) -> Eval74/1(In1)
  M075/2(LL2) -> Eval74/2(In2)
  Eval74/1(Out1) -> To Workspace74/1
  [in1] -> M076/1(CT1)
  [in2] -> M076/2(F1)
  [in3] -> M076/3(E1)
  [in4] -> M076/4(MR1)
  [in5] -> M076/5(T1)
  [in6] -> M076/6(EB1)
  [in7] -> M076/7(CT2)
  [in8] -> M076/8(F2)
  [in9] -> M076/9(E2)
  [in10] -> M076/10(MR2)
  [in11] -> M076/11(T2)
  [in12] -> M076/12(EB2)
  M076/1(LL1) -> Eval75/1(In1)
  M076/2(LL2) -> Eval75/2(In2)
  Eval75/1(Out1) -> To Workspace75/1
  [in1] -> M077/1(CT1)
  [in2] -> M077/2(F1)
  [in3] -> M077/3(E1)
  [in4] -> M077/4(MR1)
  [in5] -> M077/5(T1)
  [in6] -> M077/6(EB1)
  [in7] -> M077/7(CT2)
  [in8] -> M077/8(F2)
  [in9] -> M077/9(E2)
  [in10] -> M077/10(MR2)
  [in11] -> M077/11(T2)
  [in12] -> M077/12(EB2)
  M077/1(LL1) -> Eval76/1(In1)
  M077/2(LL2) -> Eval76/2(In2)
  Eval76/1(Out1) -> To Workspace76/1
  [in1] -> M078/1(CT1)
  [in2] -> M078/2(F1)
  [in3] -> M078/3(E1)
  [in4] -> M078/4(MR1)
  [in5] -> M078/5(T1)
  [in6] -> M078/6(EB1)
  [in7] -> M078/7(CT2)
  [in8] -> M078/8(F2)
  [in9] -> M078/9(E2)
  [in10] -> M078/10(MR2)
  [in11] -> M078/11(T2)
  [in12] -> M078/12(EB2)
  M078/1(LL1) -> Eval77/1(In1)
  M078/2(LL2) -> Eval77/2(In2)
  Eval77/1(Out1) -> To Workspace77/1
  [in1] -> M079/1(CT1)
  [in2] -> M079/2(F1)
  [in3] -> M079/3(E1)
  [in4] -> M079/4(MR1)
  [in5] -> M079/5(T1)
  [in6] -> M079/6(EB1)
  [in7] -> M079/7(CT2)
  [in8] -> M079/8(F2)
  [in9] -> M079/9(E2)
  [in10] -> M079/10(MR2)
  [in11] -> M079/11(T2)
  [in12] -> M079/12(EB2)
  M079/1(LL1) -> Eval78/1(In1)
  M079/2(LL2) -> Eval78/2(In2)
  Eval78/1(Out1) -> To Workspace78/1
  [in1] -> M080/1(CT1)
  [in2] -> M080/2(F1)
  [in3] -> M080/3(E1)
  [in4] -> M080/4(MR1)
  [in5] -> M080/5(T1)
  [in6] -> M080/6(EB1)
  [in7] -> M080/7(CT2)
  [in8] -> M080/8(F2)
  [in9] -> M080/9(E2)
  [in10] -> M080/10(MR2)
  [in11] -> M080/11(T2)
  [in12] -> M080/12(EB2)
  M080/1(LL1) -> Eval79/1(In1)
  M080/2(LL2) -> Eval79/2(In2)
  Eval79/1(Out1) -> To Workspace79/1
  [in1] -> M081/1(CT1)
  [in2] -> M081/2(F1)
  [in3] -> M081/3(E1)
  [in4] -> M081/4(MR1)
  [in5] -> M081/5(T1)
  [in6] -> M081/6(EB1)
  [in7] -> M081/7(CT2)
  [in8] -> M081/8(F2)
  [in9] -> M081/9(E2)
  [in10] -> M081/10(MR2)
  [in11] -> M081/11(T2)
  [in12] -> M081/12(EB2)
  M081/1(LL1) -> Eval80/1(In1)
  M081/2(LL2) -> Eval80/2(In2)
  Eval80/1(Out1) -> To Workspace80/1
  [in1] -> M082/1(CT1)
  [in2] -> M082/2(F1)
  [in3] -> M082/3(E1)
  [in4] -> M082/4(MR1)
  [in5] -> M082/5(T1)
  [in6] -> M082/6(EB1)
  [in7] -> M082/7(CT2)
  [in8] -> M082/8(F2)
  [in9] -> M082/9(E2)
  [in10] -> M082/10(MR2)
  [in11] -> M082/11(T2)
  [in12] -> M082/12(EB2)
  M082/1(LL1) -> Eval81/1(In1)
  M082/2(LL2) -> Eval81/2(In2)
  Eval81/1(Out1) -> To Workspace81/1
  [in1] -> M083/1(CT1)
  [in2] -> M083/2(F1)
  [in3] -> M083/3(E1)
  [in4] -> M083/4(MR1)
  [in5] -> M083/5(T1)
  [in6] -> M083/6(EB1)
  [in7] -> M083/7(CT2)
  [in8] -> M083/8(F2)
  [in9] -> M083/9(E2)
  [in10] -> M083/10(MR2)
  [in11] -> M083/11(T2)
  [in12] -> M083/12(EB2)
  M083/1(LL1) -> Eval82/1(In1)
  M083/2(LL2) -> Eval82/2(In2)
  Eval82/1(Out1) -> To Workspace82/1
  [in1] -> M118/1(CT1)
  [in2] -> M118/2(F1)
  [in3] -> M118/3(E1)
  [in4] -> M118/4(MR1)
  [in5] -> M118/5(T1)
  [in6] -> M118/6(EB1)
  [in7] -> M118/7(CT2)
  [in8] -> M118/8(F2)
  [in9] -> M118/9(E2)
  [in10] -> M118/10(MR2)
  [in11] -> M118/11(T2)
  [in12] -> M118/12(EB2)
  M118/1(LL1) -> Eval117/1(In1)
  M118/2(LL2) -> Eval117/2(In2)
  Eval117/1(Out1) -> To Workspace117/1
  [in1] -> M119/1(CT1)
  [in2] -> M119/2(F1)
  [in3] -> M119/3(E1)
  [in4] -> M119/4(MR1)
  [in5] -> M119/5(T1)
  [in6] -> M119/6(EB1)
  [in7] -> M119/7(CT2)
  [in8] -> M119/8(F2)
  [in9] -> M119/9(E2)
  [in10] -> M119/10(MR2)
  [in11] -> M119/11(T2)
  [in12] -> M119/12(EB2)
  M119/1(LL1) -> Eval118/1(In1)
  M119/2(LL2) -> Eval118/2(In2)
  Eval118/1(Out1) -> To Workspace118/1
  [in1] -> M120/1(CT1)
  [in2] -> M120/2(F1)
  [in3] -> M120/3(E1)
  [in4] -> M120/4(MR1)
  [in5] -> M120/5(T1)
  [in6] -> M120/6(EB1)
  [in7] -> M120/7(CT2)
  [in8] -> M120/8(F2)
  [in9] -> M120/9(E2)
  [in10] -> M120/10(MR2)
  [in11] -> M120/11(T2)
  [in12] -> M120/12(EB2)
  M120/1(LL1) -> Eval119/1(In1)
  M120/2(LL2) -> Eval119/2(In2)
  Eval119/1(Out1) -> To Workspace119/1
  [in1] -> M121/1(CT1)
  [in2] -> M121/2(F1)
  [in3] -> M121/3(E1)
  [in4] -> M121/4(MR1)
  [in5] -> M121/5(T1)
  [in6] -> M121/6(EB1)
  [in7] -> M121/7(CT2)
  [in8] -> M121/8(F2)
  [in9] -> M121/9(E2)
  [in10] -> M121/10(MR2)
  [in11] -> M121/11(T2)
  [in12] -> M121/12(EB2)
  M121/1(LL1) -> Eval120/1(In1)
  M121/2(LL2) -> Eval120/2(In2)
  Eval120/1(Out1) -> To Workspace120/1
  [in1] -> M122/1(CT1)
  [in2] -> M122/2(F1)
  [in3] -> M122/3(E1)
  [in4] -> M122/4(MR1)
  [in5] -> M122/5(T1)
  [in6] -> M122/6(EB1)
  [in7] -> M122/7(CT2)
  [in8] -> M122/8(F2)
  [in9] -> M122/9(E2)
  [in10] -> M122/10(MR2)
  [in11] -> M122/11(T2)
  [in12] -> M122/12(EB2)
  M122/1(LL1) -> Eval121/1(In1)
  M122/2(LL2) -> Eval121/2(In2)
  Eval121/1(Out1) -> To Workspace121/1
  [in1] -> M123/1(CT1)
  [in2] -> M123/2(F1)
  [in3] -> M123/3(E1)
  [in4] -> M123/4(MR1)
  [in5] -> M123/5(T1)
  [in6] -> M123/6(EB1)
  [in7] -> M123/7(CT2)
  [in8] -> M123/8(F2)
  [in9] -> M123/9(E2)
  [in10] -> M123/10(MR2)
  [in11] -> M123/11(T2)
  [in12] -> M123/12(EB2)
  M123/1(LL1) -> Eval122/1(In1)
  M123/2(LL2) -> Eval122/2(In2)
  Eval122/1(Out1) -> To Workspace122/1
  [in1] -> M124/1(CT1)
  [in2] -> M124/2(F1)
  [in3] -> M124/3(E1)
  [in4] -> M124/4(MR1)
  [in5] -> M124/5(T1)
  [in6] -> M124/6(EB1)
  [in7] -> M124/7(CT2)
  [in8] -> M124/8(F2)
  [in9] -> M124/9(E2)
  [in10] -> M124/10(MR2)
  [in11] -> M124/11(T2)
  [in12] -> M124/12(EB2)
  M124/1(LL1) -> Eval123/1(In1)
  M124/2(LL2) -> Eval123/2(In2)
  Eval123/1(Out1) -> To Workspace123/1
  [in1] -> M125/1(CT1)
  [in2] -> M125/2(F1)
  [in3] -> M125/3(E1)
  [in4] -> M125/4(MR1)
  [in5] -> M125/5(T1)
  [in6] -> M125/6(EB1)
  [in7] -> M125/7(CT2)
  [in8] -> M125/8(F2)
  [in9] -> M125/9(E2)
  [in10] -> M125/10(MR2)
  [in11] -> M125/11(T2)
  [in12] -> M125/12(EB2)
  M125/1(LL1) -> Eval124/1(In1)
  M125/2(LL2) -> Eval124/2(In2)
  Eval124/1(Out1) -> To Workspace124/1
  [in1] -> M126/1(CT1)
  [in2] -> M126/2(F1)
  [in3] -> M126/3(E1)
  [in4] -> M126/4(MR1)
  [in5] -> M126/5(T1)
  [in6] -> M126/6(EB1)
  [in7] -> M126/7(CT2)
  [in8] -> M126/8(F2)
  [in9] -> M126/9(E2)
  [in10] -> M126/10(MR2)
  [in11] -> M126/11(T2)
  [in12] -> M126/12(EB2)
  M126/1(LL1) -> Eval125/1(In1)
  M126/2(LL2) -> Eval125/2(In2)
  Eval125/1(Out1) -> To Workspace125/1
  [in1] -> M127/1(CT1)
  [in2] -> M127/2(F1)
  [in3] -> M127/3(E1)
  [in4] -> M127/4(MR1)
  [in5] -> M127/5(T1)
  [in6] -> M127/6(EB1)
  [in7] -> M127/7(CT2)
  [in8] -> M127/8(F2)
  [in9] -> M127/9(E2)
  [in10] -> M127/10(MR2)
  [in11] -> M127/11(T2)
  [in12] -> M127/12(EB2)
  M127/1(LL1) -> Eval126/1(In1)
  M127/2(LL2) -> Eval126/2(In2)
  Eval126/1(Out1) -> To Workspace126/1
  [in1] -> M128/1(CT1)
  [in2] -> M128/2(F1)
  [in3] -> M128/3(E1)
  [in4] -> M128/4(MR1)
  [in5] -> M128/5(T1)
  [in6] -> M128/6(EB1)
  [in7] -> M128/7(CT2)
  [in8] -> M128/8(F2)
  [in9] -> M128/9(E2)
  [in10] -> M128/10(MR2)
  [in11] -> M128/11(T2)
  [in12] -> M128/12(EB2)
  M128/1(LL1) -> Eval127/1(In1)
  M128/2(LL2) -> Eval127/2(In2)
  Eval127/1(Out1) -> To Workspace127/1
  [in1] -> M129/1(CT1)
  [in2] -> M129/2(F1)
  [in3] -> M129/3(E1)
  [in4] -> M129/4(MR1)
  [in5] -> M129/5(T1)
  [in6] -> M129/6(EB1)
  [in7] -> M129/7(CT2)
  [in8] -> M129/8(F2)
  [in9] -> M129/9(E2)
  [in10] -> M129/10(MR2)
  [in11] -> M129/11(T2)
  [in12] -> M129/12(EB2)
  M129/1(LL1) -> Eval128/1(In1)
  M129/2(LL2) -> Eval128/2(In2)
  Eval128/1(Out1) -> To Workspace128/1
  [in1] -> M130/1(CT1)
  [in2] -> M130/2(F1)
  [in3] -> M130/3(E1)
  [in4] -> M130/4(MR1)
  [in5] -> M130/5(T1)
  [in6] -> M130/6(EB1)
  [in7] -> M130/7(CT2)
  [in8] -> M130/8(F2)
  [in9] -> M130/9(E2)
  [in10] -> M130/10(MR2)
  [in11] -> M130/11(T2)
  [in12] -> M130/12(EB2)
  M130/1(LL1) -> Eval129/1(In1)
  M130/2(LL2) -> Eval129/2(In2)
  Eval129/1(Out1) -> To Workspace129/1
  [in1] -> M131/1(CT1)
  [in2] -> M131/2(F1)
  [in3] -> M131/3(E1)
  [in4] -> M131/4(MR1)
  [in5] -> M131/5(T1)
  [in6] -> M131/6(EB1)
  [in7] -> M131/7(CT2)
  [in8] -> M131/8(F2)
  [in9] -> M131/9(E2)
  [in10] -> M131/10(MR2)
  [in11] -> M131/11(T2)
  [in12] -> M131/12(EB2)
  M131/1(LL1) -> Eval130/1(In1)
  M131/2(LL2) -> Eval130/2(In2)
  Eval130/1(Out1) -> To Workspace130/1
  [in1] -> M132/1(CT1)
  [in2] -> M132/2(F1)
  [in3] -> M132/3(E1)
  [in4] -> M132/4(MR1)
  [in5] -> M132/5(T1)
  [in6] -> M132/6(EB1)
  [in7] -> M132/7(CT2)
  [in8] -> M132/8(F2)
  [in9] -> M132/9(E2)
  [in10] -> M132/10(MR2)
  [in11] -> M132/11(T2)
  [in12] -> M132/12(EB2)
  M132/1(LL1) -> Eval131/1(In1)
  M132/2(LL2) -> Eval131/2(In2)
  Eval131/1(Out1) -> To Workspace131/1
  [in1] -> M133/1(CT1)
  [in2] -> M133/2(F1)
  [in3] -> M133/3(E1)
  [in4] -> M133/4(MR1)
  [in5] -> M133/5(T1)
  [in6] -> M133/6(EB1)
  [in7] -> M133/7(CT2)
  [in8] -> M133/8(F2)
  [in9] -> M133/9(E2)
  [in10] -> M133/10(MR2)
  [in11] -> M133/11(T2)
  [in12] -> M133/12(EB2)
  M133/1(LL1) -> Eval132/1(In1)
  M133/2(LL2) -> Eval132/2(In2)
  Eval132/1(Out1) -> To Workspace132/1
  [in1] -> M134/1(CT1)
  [in2] -> M134/2(F1)
  [in3] -> M134/3(E1)
  [in4] -> M134/4(MR1)
  [in5] -> M134/5(T1)
  [in6] -> M134/6(EB1)
  [in7] -> M134/7(CT2)
  [in8] -> M134/8(F2)
  [in9] -> M134/9(E2)
  [in10] -> M134/10(MR2)
  [in11] -> M134/11(T2)
  [in12] -> M134/12(EB2)
  M134/1(LL1) -> Eval133/1(In1)
  M134/2(LL2) -> Eval133/2(In2)
  Eval133/1(Out1) -> To Workspace133/1
  [in1] -> M135/1(CT1)
  [in2] -> M135/2(F1)
  [in3] -> M135/3(E1)
  [in4] -> M135/4(MR1)
  [in5] -> M135/5(T1)
  [in6] -> M135/6(EB1)
  [in7] -> M135/7(CT2)
  [in8] -> M135/8(F2)
  [in9] -> M135/9(E2)
  [in10] -> M135/10(MR2)
  [in11] -> M135/11(T2)
  [in12] -> M135/12(EB2)
  M135/1(LL1) -> Eval134/1(In1)
  M135/2(LL2) -> Eval134/2(In2)
  Eval134/1(Out1) -> To Workspace134/1
  [in1] -> M136/1(CT1)
  [in2] -> M136/2(F1)
  [in3] -> M136/3(E1)
  [in4] -> M136/4(MR1)
  [in5] -> M136/5(T1)
  [in6] -> M136/6(EB1)
  [in7] -> M136/7(CT2)
  [in8] -> M136/8(F2)
  [in9] -> M136/9(E2)
  [in10] -> M136/10(MR2)
  [in11] -> M136/11(T2)
  [in12] -> M136/12(EB2)
  M136/1(LL1) -> Eval135/1(In1)
  M136/2(LL2) -> Eval135/2(In2)
  Eval135/1(Out1) -> To Workspace135/1
  [in1] -> M137/1(CT1)
  [in2] -> M137/2(F1)
  [in3] -> M137/3(E1)
  [in4] -> M137/4(MR1)
  [in5] -> M137/5(T1)
  [in6] -> M137/6(EB1)
  [in7] -> M137/7(CT2)
  [in8] -> M137/8(F2)
  [in9] -> M137/9(E2)
  [in10] -> M137/10(MR2)
  [in11] -> M137/11(T2)
  [in12] -> M137/12(EB2)
  M137/1(LL1) -> Eval136/1(In1)
  M137/2(LL2) -> Eval136/2(In2)
  Eval136/1(Out1) -> To Workspace136/1
  [in1] -> M138/1(CT1)
  [in2] -> M138/2(F1)
  [in3] -> M138/3(E1)
  [in4] -> M138/4(MR1)
  [in5] -> M138/5(T1)
  [in6] -> M138/6(EB1)
  [in7] -> M138/7(CT2)
  [in8] -> M138/8(F2)
  [in9] -> M138/9(E2)
  [in10] -> M138/10(MR2)
  [in11] -> M138/11(T2)
  [in12] -> M138/12(EB2)
  M138/1(LL1) -> Eval137/1(In1)
  M138/2(LL2) -> Eval137/2(In2)
  Eval137/1(Out1) -> To Workspace137/1
  [in1] -> M140/1(CT1)
  [in2] -> M140/2(F1)
  [in3] -> M140/3(E1)
  [in4] -> M140/4(MR1)
  [in5] -> M140/5(T1)
  [in6] -> M140/6(EB1)
  [in7] -> M140/7(CT2)
  [in8] -> M140/8(F2)
  [in9] -> M140/9(E2)
  [in10] -> M140/10(MR2)
  [in11] -> M140/11(T2)
  [in12] -> M140/12(EB2)
  M140/1(LL1) -> Eval139/1(In1)
  M140/2(LL2) -> Eval139/2(In2)
  Eval139/1(Out1) -> To Workspace139/1
  [in1] -> M141/1(CT1)
  [in2] -> M141/2(F1)
  [in3] -> M141/3(E1)
  [in4] -> M141/4(MR1)
  [in5] -> M141/5(T1)
  [in6] -> M141/6(EB1)
  [in7] -> M141/7(CT2)
  [in8] -> M141/8(F2)
  [in9] -> M141/9(E2)
  [in10] -> M141/10(MR2)
  [in11] -> M141/11(T2)
  [in12] -> M141/12(EB2)
  M141/1(LL1) -> Eval140/1(In1)
  M141/2(LL2) -> Eval140/2(In2)
  Eval140/1(Out1) -> To Workspace140/1
  [in1] -> M142/1(CT1)
  [in2] -> M142/2(F1)
  [in3] -> M142/3(E1)
  [in4] -> M142/4(MR1)
  [in5] -> M142/5(T1)
  [in6] -> M142/6(EB1)
  [in7] -> M142/7(CT2)
  [in8] -> M142/8(F2)
  [in9] -> M142/9(E2)
  [in10] -> M142/10(MR2)
  [in11] -> M142/11(T2)
  [in12] -> M142/12(EB2)
  M142/1(LL1) -> Eval141/1(In1)
  M142/2(LL2) -> Eval141/2(In2)
  Eval141/1(Out1) -> To Workspace141/1
  [in1] -> M143/1(CT1)
  [in2] -> M143/2(F1)
  [in3] -> M143/3(E1)
  [in4] -> M143/4(MR1)
  [in5] -> M143/5(T1)
  [in6] -> M143/6(EB1)
  [in7] -> M143/7(CT2)
  [in8] -> M143/8(F2)
  [in9] -> M143/9(E2)
  [in10] -> M143/10(MR2)
  [in11] -> M143/11(T2)
  [in12] -> M143/12(EB2)
  M143/1(LL1) -> Eval142/1(In1)
  M143/2(LL2) -> Eval142/2(In2)
  Eval142/1(Out1) -> To Workspace142/1
  [in1] -> M144/1(CT1)
  [in2] -> M144/2(F1)
  [in3] -> M144/3(E1)
  [in4] -> M144/4(MR1)
  [in5] -> M144/5(T1)
  [in6] -> M144/6(EB1)
  [in7] -> M144/7(CT2)
  [in8] -> M144/8(F2)
  [in9] -> M144/9(E2)
  [in10] -> M144/10(MR2)
  [in11] -> M144/11(T2)
  [in12] -> M144/12(EB2)
  M144/1(LL1) -> Eval143/1(In1)
  M144/2(LL2) -> Eval143/2(In2)
  Eval143/1(Out1) -> To Workspace143/1
  [in1] -> M145/1(CT1)
  [in2] -> M145/2(F1)
  [in3] -> M145/3(E1)
  [in4] -> M145/4(MR1)
  [in5] -> M145/5(T1)
  [in6] -> M145/6(EB1)
  [in7] -> M145/7(CT2)
  [in8] -> M145/8(F2)
  [in9] -> M145/9(E2)
  [in10] -> M145/10(MR2)
  [in11] -> M145/11(T2)
  [in12] -> M145/12(EB2)
  M145/1(LL1) -> Eval144/1(In1)
  M145/2(LL2) -> Eval144/2(In2)
  Eval144/1(Out1) -> To Workspace144/1
  [in1] -> M146/1(CT1)
  [in2] -> M146/2(F1)
  [in3] -> M146/3(E1)
  [in4] -> M146/4(MR1)
  [in5] -> M146/5(T1)
  [in6] -> M146/6(EB1)
  [in7] -> M146/7(CT2)
  [in8] -> M146/8(F2)
  [in9] -> M146/9(E2)
  [in10] -> M146/10(MR2)
  [in11] -> M146/11(T2)
  [in12] -> M146/12(EB2)
  M146/1(LL1) -> Eval145/1(In1)
  M146/2(LL2) -> Eval145/2(In2)
  Eval145/1(Out1) -> To Workspace145/1
  [in1] -> M147/1(CT1)
  [in2] -> M147/2(F1)
  [in3] -> M147/3(E1)
  [in4] -> M147/4(MR1)
  [in5] -> M147/5(T1)
  [in6] -> M147/6(EB1)
  [in7] -> M147/7(CT2)
  [in8] -> M147/8(F2)
  [in9] -> M147/9(E2)
  [in10] -> M147/10(MR2)
  [in11] -> M147/11(T2)
  [in12] -> M147/12(EB2)
  M147/1(LL1) -> Eval146/1(In1)
  M147/2(LL2) -> Eval146/2(In2)
  Eval146/1(Out1) -> To Workspace146/1
  [in1] -> M148/1(CT1)
  [in2] -> M148/2(F1)
  [in3] -> M148/3(E1)
  [in4] -> M148/4(MR1)
  [in5] -> M148/5(T1)
  [in6] -> M148/6(EB1)
  [in7] -> M148/7(CT2)
  [in8] -> M148/8(F2)
  [in9] -> M148/9(E2)
  [in10] -> M148/10(MR2)
  [in11] -> M148/11(T2)
  [in12] -> M148/12(EB2)
  M148/1(LL1) -> Eval147/1(In1)
  M148/2(LL2) -> Eval147/2(In2)
  Eval147/1(Out1) -> To Workspace147/1
  [in1] -> M149/1(CT1)
  [in2] -> M149/2(F1)
  [in3] -> M149/3(E1)
  [in4] -> M149/4(MR1)
  [in5] -> M149/5(T1)
  [in6] -> M149/6(EB1)
  [in7] -> M149/7(CT2)
  [in8] -> M149/8(F2)
  [in9] -> M149/9(E2)
  [in10] -> M149/10(MR2)
  [in11] -> M149/11(T2)
  [in12] -> M149/12(EB2)
  M149/1(LL1) -> Eval148/1(In1)
  M149/2(LL2) -> Eval148/2(In2)
  Eval148/1(Out1) -> To Workspace148/1
  [in1] -> M150/1(CT1)
  [in2] -> M150/2(F1)
  [in3] -> M150/3(E1)
  [in4] -> M150/4(MR1)
  [in5] -> M150/5(T1)
  [in6] -> M150/6(EB1)
  [in7] -> M150/7(CT2)
  [in8] -> M150/8(F2)
  [in9] -> M150/9(E2)
  [in10] -> M150/10(MR2)
  [in11] -> M150/11(T2)
  [in12] -> M150/12(EB2)
  M150/1(LL1) -> Eval149/1(In1)
  M150/2(LL2) -> Eval149/2(In2)
  Eval149/1(Out1) -> To Workspace149/1
  [in1] -> M151/1(CT1)
  [in2] -> M151/2(F1)
  [in3] -> M151/3(E1)
  [in4] -> M151/4(MR1)
  [in5] -> M151/5(T1)
  [in6] -> M151/6(EB1)
  [in7] -> M151/7(CT2)
  [in8] -> M151/8(F2)
  [in9] -> M151/9(E2)
  [in10] -> M151/10(MR2)
  [in11] -> M151/11(T2)
  [in12] -> M151/12(EB2)
  M151/1(LL1) -> Eval150/1(In1)
  M151/2(LL2) -> Eval150/2(In2)
  Eval150/1(Out1) -> To Workspace150/1
  [in1] -> M152/1(CT1)
  [in2] -> M152/2(F1)
  [in3] -> M152/3(E1)
  [in4] -> M152/4(MR1)
  [in5] -> M152/5(T1)
  [in6] -> M152/6(EB1)
  [in7] -> M152/7(CT2)
  [in8] -> M152/8(F2)
  [in9] -> M152/9(E2)
  [in10] -> M152/10(MR2)
  [in11] -> M152/11(T2)
  [in12] -> M152/12(EB2)
  M152/1(LL1) -> Eval151/1(In1)
  M152/2(LL2) -> Eval151/2(In2)
  Eval151/1(Out1) -> To Workspace151/1
  [in1] -> M153/1(CT1)
  [in2] -> M153/2(F1)
  [in3] -> M153/3(E1)
  [in4] -> M153/4(MR1)
  [in5] -> M153/5(T1)
  [in6] -> M153/6(EB1)
  [in7] -> M153/7(CT2)
  [in8] -> M153/8(F2)
  [in9] -> M153/9(E2)
  [in10] -> M153/10(MR2)
  [in11] -> M153/11(T2)
  [in12] -> M153/12(EB2)
  M153/1(LL1) -> Eval152/1(In1)
  M153/2(LL2) -> Eval152/2(In2)
  Eval152/1(Out1) -> To Workspace152/1
  [in1] -> M154/1(CT1)
  [in2] -> M154/2(F1)
  [in3] -> M154/3(E1)
  [in4] -> M154/4(MR1)
  [in5] -> M154/5(T1)
  [in6] -> M154/6(EB1)
  [in7] -> M154/7(CT2)
  [in8] -> M154/8(F2)
  [in9] -> M154/9(E2)
  [in10] -> M154/10(MR2)
  [in11] -> M154/11(T2)
  [in12] -> M154/12(EB2)
  M154/1(LL1) -> Eval153/1(In1)
  M154/2(LL2) -> Eval153/2(In2)
  Eval153/1(Out1) -> To Workspace153/1
  [in1] -> M155/1(CT1)
  [in2] -> M155/2(F1)
  [in3] -> M155/3(E1)
  [in4] -> M155/4(MR1)
  [in5] -> M155/5(T1)
  [in6] -> M155/6(EB1)
  [in7] -> M155/7(CT2)
  [in8] -> M155/8(F2)
  [in9] -> M155/9(E2)
  [in10] -> M155/10(MR2)
  [in11] -> M155/11(T2)
  [in12] -> M155/12(EB2)
  M155/1(LL1) -> Eval154/1(In1)
  M155/2(LL2) -> Eval154/2(In2)
  Eval154/1(Out1) -> To Workspace154/1
  [in1] -> M156/1(CT1)
  [in2] -> M156/2(F1)
  [in3] -> M156/3(E1)
  [in4] -> M156/4(MR1)
  [in5] -> M156/5(T1)
  [in6] -> M156/6(EB1)
  [in7] -> M156/7(CT2)
  [in8] -> M156/8(F2)
  [in9] -> M156/9(E2)
  [in10] -> M156/10(MR2)
  [in11] -> M156/11(T2)
  [in12] -> M156/12(EB2)
  M156/1(LL1) -> Eval155/1(In1)
  M156/2(LL2) -> Eval155/2(In2)
  Eval155/1(Out1) -> To Workspace155/1
  [in1] -> M157/1(CT1)
  [in2] -> M157/2(F1)
  [in3] -> M157/3(E1)
  [in4] -> M157/4(MR1)
  [in5] -> M157/5(T1)
  [in6] -> M157/6(EB1)
  [in7] -> M157/7(CT2)
  [in8] -> M157/8(F2)
  [in9] -> M157/9(E2)
  [in10] -> M157/10(MR2)
  [in11] -> M157/11(T2)
  [in12] -> M157/12(EB2)
  M157/1(LL1) -> Eval156/1(In1)
  M157/2(LL2) -> Eval156/2(In2)
  Eval156/1(Out1) -> To Workspace156/1
  [in1] -> M158/1(CT1)
  [in2] -> M158/2(F1)
  [in3] -> M158/3(E1)
  [in4] -> M158/4(MR1)
  [in5] -> M158/5(T1)
  [in6] -> M158/6(EB1)
  [in7] -> M158/7(CT2)
  [in8] -> M158/8(F2)
  [in9] -> M158/9(E2)
  [in10] -> M158/10(MR2)
  [in11] -> M158/11(T2)
  [in12] -> M158/12(EB2)
  M158/1(LL1) -> Eval157/1(In1)
  M158/2(LL2) -> Eval157/2(In2)
  Eval157/1(Out1) -> To Workspace157/1
  [in1] -> M159/1(CT1)
  [in2] -> M159/2(F1)
  [in3] -> M159/3(E1)
  [in4] -> M159/4(MR1)
  [in5] -> M159/5(T1)
  [in6] -> M159/6(EB1)
  [in7] -> M159/7(CT2)
  [in8] -> M159/8(F2)
  [in9] -> M159/9(E2)
  [in10] -> M159/10(MR2)
  [in11] -> M159/11(T2)
  [in12] -> M159/12(EB2)
  M159/1(LL1) -> Eval158/1(In1)
  M159/2(LL2) -> Eval158/2(In2)
  Eval158/1(Out1) -> To Workspace158/1
  [in1] -> M160/1(CT1)
  [in2] -> M160/2(F1)
  [in3] -> M160/3(E1)
  [in4] -> M160/4(MR1)
  [in5] -> M160/5(T1)
  [in6] -> M160/6(EB1)
  [in7] -> M160/7(CT2)
  [in8] -> M160/8(F2)
  [in9] -> M160/9(E2)
  [in10] -> M160/10(MR2)
  [in11] -> M160/11(T2)
  [in12] -> M160/12(EB2)
  M160/1(LL1) -> Eval159/1(In1)
  M160/2(LL2) -> Eval159/2(In2)
  Eval159/1(Out1) -> To Workspace159/1
  [in1] -> M161/1(CT1)
  [in2] -> M161/2(F1)
  [in3] -> M161/3(E1)
  [in4] -> M161/4(MR1)
  [in5] -> M161/5(T1)
  [in6] -> M161/6(EB1)
  [in7] -> M161/7(CT2)
  [in8] -> M161/8(F2)
  [in9] -> M161/9(E2)
  [in10] -> M161/10(MR2)
  [in11] -> M161/11(T2)
  [in12] -> M161/12(EB2)
  M161/1(LL1) -> Eval160/1(In1)
  M161/2(LL2) -> Eval160/2(In2)
  Eval160/1(Out1) -> To Workspace160/1
  [in1] -> M162/1(CT1)
  [in2] -> M162/2(F1)
  [in3] -> M162/3(E1)
  [in4] -> M162/4(MR1)
  [in5] -> M162/5(T1)
  [in6] -> M162/6(EB1)
  [in7] -> M162/7(CT2)
  [in8] -> M162/8(F2)
  [in9] -> M162/9(E2)
  [in10] -> M162/10(MR2)
  [in11] -> M162/11(T2)
  [in12] -> M162/12(EB2)
  M162/1(LL1) -> Eval161/1(In1)
  M162/2(LL2) -> Eval161/2(In2)
  Eval161/1(Out1) -> To Workspace161/1
  [in1] -> M163/1(CT1)
  [in2] -> M163/2(F1)
  [in3] -> M163/3(E1)
  [in4] -> M163/4(MR1)
  [in5] -> M163/5(T1)
  [in6] -> M163/6(EB1)
  [in7] -> M163/7(CT2)
  [in8] -> M163/8(F2)
  [in9] -> M163/9(E2)
  [in10] -> M163/10(MR2)
  [in11] -> M163/11(T2)
  [in12] -> M163/12(EB2)
  M163/1(LL1) -> Eval162/1(In1)
  M163/2(LL2) -> Eval162/2(In2)
  Eval162/1(Out1) -> To Workspace162/1
  [in1] -> M164/1(CT1)
  [in2] -> M164/2(F1)
  [in3] -> M164/3(E1)
  [in4] -> M164/4(MR1)
  [in5] -> M164/5(T1)
  [in6] -> M164/6(EB1)
  [in7] -> M164/7(CT2)
  [in8] -> M164/8(F2)
  [in9] -> M164/9(E2)
  [in10] -> M164/10(MR2)
  [in11] -> M164/11(T2)
  [in12] -> M164/12(EB2)
  M164/1(LL1) -> Eval163/1(In1)
  M164/2(LL2) -> Eval163/2(In2)
  Eval163/1(Out1) -> To Workspace163/1
  [in1] -> M226/1(CT1)
  [in2] -> M226/2(F1)
  [in3] -> M226/3(E1)
  [in4] -> M226/4(MR1)
  [in5] -> M226/5(T1)
  [in6] -> M226/6(EB1)
  [in7] -> M226/7(CT2)
  [in8] -> M226/8(F2)
  [in9] -> M226/9(E2)
  [in10] -> M226/10(MR2)
  [in11] -> M226/11(T2)
  [in12] -> M226/12(EB2)
  M226/1(LL1) -> Eval225/1(In1)
  M226/2(LL2) -> Eval225/2(In2)
  Eval225/1(Out1) -> To Workspace225/1
  [in1] -> M227/1(CT1)
  [in2] -> M227/2(F1)
  [in3] -> M227/3(E1)
  [in4] -> M227/4(MR1)
  [in5] -> M227/5(T1)
  [in6] -> M227/6(EB1)
  [in7] -> M227/7(CT2)
  [in8] -> M227/8(F2)
  [in9] -> M227/9(E2)
  [in10] -> M227/10(MR2)
  [in11] -> M227/11(T2)
  [in12] -> M227/12(EB2)
  M227/1(LL1) -> Eval226/1(In1)
  M227/2(LL2) -> Eval226/2(In2)
  Eval226/1(Out1) -> To Workspace226/1
  [in1] -> M228/1(CT1)
  [in2] -> M228/2(F1)
  [in3] -> M228/3(E1)
  [in4] -> M228/4(MR1)
  [in5] -> M228/5(T1)
  [in6] -> M228/6(EB1)
  [in7] -> M228/7(CT2)
  [in8] -> M228/8(F2)
  [in9] -> M228/9(E2)
  [in10] -> M228/10(MR2)
  [in11] -> M228/11(T2)
  [in12] -> M228/12(EB2)
  M228/1(LL1) -> Eval227/1(In1)
  M228/2(LL2) -> Eval227/2(In2)
  Eval227/1(Out1) -> To Workspace227/1
  [in1] -> M229/1(CT1)
  [in2] -> M229/2(F1)
  [in3] -> M229/3(E1)
  [in4] -> M229/4(MR1)
  [in5] -> M229/5(T1)
  [in6] -> M229/6(EB1)
  [in7] -> M229/7(CT2)
  [in8] -> M229/8(F2)
  [in9] -> M229/9(E2)
  [in10] -> M229/10(MR2)
  [in11] -> M229/11(T2)
  [in12] -> M229/12(EB2)
  M229/1(LL1) -> Eval228/1(In1)
  M229/2(LL2) -> Eval228/2(In2)
  Eval228/1(Out1) -> To Workspace228/1
  [in1] -> M230/1(CT1)
  [in2] -> M230/2(F1)
  [in3] -> M230/3(E1)
  [in4] -> M230/4(MR1)
  [in5] -> M230/5(T1)
  [in6] -> M230/6(EB1)
  [in7] -> M230/7(CT2)
  [in8] -> M230/8(F2)
  [in9] -> M230/9(E2)
  [in10] -> M230/10(MR2)
  [in11] -> M230/11(T2)
  [in12] -> M230/12(EB2)
  M230/1(LL1) -> Eval229/1(In1)
  M230/2(LL2) -> Eval229/2(In2)
  Eval229/1(Out1) -> To Workspace229/1
  Inputs/1(CT1) -> dtc_CT1/1
  dtc_CT1/1 -> CPSUT/1(CT1), [in1]
  Inputs/2(F1) -> dtc_F1/1
  dtc_F1/1 -> CPSUT/2(F1), [in2]
  Inputs/3(E1) -> dtc_E1/1
  dtc_E1/1 -> CPSUT/3(E1), [in3]
  Inputs/4(MR1) -> dtc_MR1/1
  dtc_MR1/1 -> CPSUT/4(MR1), [in4]
  Inputs/5(T1) -> dtc_T1/1
  dtc_T1/1 -> [in5]
  Inputs/6(EB1) -> dtc_EB1/1
  dtc_EB1/1 -> CPSUT/5(EB1), [in6]
  Inputs/7(CT2) -> dtc_CT2/1
  dtc_CT2/1 -> CPSUT/6(CT2), [in7]
  Inputs/8(F2) -> dtc_F2/1
  dtc_F2/1 -> CPSUT/7(F2), [in8]
  Inputs/9(E2) -> dtc_E2/1
  dtc_E2/1 -> CPSUT/8(E2), [in9]
  Inputs/10(MR2) -> dtc_MR2/1
  dtc_MR2/1 -> CPSUT/9(MR2), [in10]
  Inputs/11(T2) -> dtc_T2/1
  dtc_T2/1 -> CPSUT/10(T2), [in11]
  Inputs/12(EB2) -> dtc_EB2/1
  dtc_EB2/1 -> CPSUT/11(EB2), [in12]
